simulink model "V3ASM"  (R2020b)
(part 12 of 23)

  Transform63 : sm_lib/Frames and Transforms/Rigid Transform  TranslationMethod=Cartesian  TranslationStandardOffset=0  TranslationLengthUnit=mm  TranslationStandardAxis=+Z  TranslationCartesianOffset=smiData.RigidTransform(303).translation  TranslationROffset=0  TranslationROffsetUnits=m  TranslationZOffset=0  TranslationZOffsetUnits=m  TranslationThetaOffset=0  TranslationThetaOffsetUnits=deg  RotationMethod=ArbitraryAxis  RotationAngleUnits=rad  RotationStandardAxis=+Z  RotationAngle=smiData.RigidTransform(303).angle  RotationArbitraryAxis=smiData.RigidTransform(303).axis  FollAlignAxisA=+X  BaseAlignAxisA=+Y  FollAlignAxisB=+Y  BaseAlignAxisB=+Z  RotationSequenceAxes=FollowerAxes  RotationSequence=XYX  RotationSequenceAngles=[0 0 0]  RotationSequenceAnglesUnits=deg  RotationMatrix=[1 0 0; 0 1 0; 0 0 1]
  Transform64 : sm_lib/Frames and Transforms/Rigid Transform  TranslationMethod=Cartesian  TranslationStandardOffset=0  TranslationLengthUnit=mm  TranslationStandardAxis=+Z  TranslationCartesianOffset=smiData.RigidTransform(304).translation  TranslationROffset=0  TranslationROffsetUnits=m  TranslationZOffset=0  TranslationZOffsetUnits=m  TranslationThetaOffset=0  TranslationThetaOffsetUnits=deg  RotationMethod=ArbitraryAxis  RotationAngleUnits=rad  RotationStandardAxis=+Z  RotationAngle=smiData.RigidTransform(304).angle  RotationArbitraryAxis=smiData.RigidTransform(304).axis  FollAlignAxisA=+X  BaseAlignAxisA=+Y  FollAlignAxisB=+Y  BaseAlignAxisB=+Z  RotationSequenceAxes=FollowerAxes  RotationSequence=XYX  RotationSequenceAngles=[0 0 0]  RotationSequenceAnglesUnits=deg  RotationMatrix=[1 0 0; 0 1 0; 0 0 1]
  Transform65 : sm_lib/Frames and Transforms/Rigid Transform  TranslationMethod=Cartesian  TranslationStandardOffset=0  TranslationLengthUnit=mm  TranslationStandardAxis=+Z  TranslationCartesianOffset=smiData.RigidTransform(305).translation  TranslationROffset=0  TranslationROffsetUnits=m  TranslationZOffset=0  TranslationZOffsetUnits=m  TranslationThetaOffset=0  TranslationThetaOffsetUnits=deg  RotationMethod=ArbitraryAxis  RotationAngleUnits=rad  RotationStandardAxis=+Z  RotationAngle=smiData.RigidTransform(305).angle  RotationArbitraryAxis=smiData.RigidTransform(305).axis  FollAlignAxisA=+X  BaseAlignAxisA=+Y  FollAlignAxisB=+Y  BaseAlignAxisB=+Z  RotationSequenceAxes=FollowerAxes  RotationSequence=XYX  RotationSequenceAngles=[0 0 0]  RotationSequenceAnglesUnits=deg  RotationMatrix=[1 0 0; 0 1 0; 0 0 1]
  Transform66 : sm_lib/Frames and Transforms/Rigid Transform  TranslationMethod=Cartesian  TranslationStandardOffset=0  TranslationLengthUnit=mm  TranslationStandardAxis=+Z  TranslationCartesianOffset=smiData.RigidTransform(306).translation  TranslationROffset=0  TranslationROffsetUnits=m  TranslationZOffset=0  TranslationZOffsetUnits=m  TranslationThetaOffset=0  TranslationThetaOffsetUnits=deg  RotationMethod=ArbitraryAxis  RotationAngleUnits=rad  RotationStandardAxis=+Z  RotationAngle=smiData.RigidTransform(306).angle  RotationArbitraryAxis=smiData.RigidTransform(306).axis  FollAlignAxisA=+X  BaseAlignAxisA=+Y  FollAlignAxisB=+Y  BaseAlignAxisB=+Z  RotationSequenceAxes=FollowerAxes  RotationSequence=XYX  RotationSequenceAngles=[0 0 0]  RotationSequenceAnglesUnits=deg  RotationMatrix=[1 0 0; 0 1 0; 0 0 1]
  Transform67 : sm_lib/Frames and Transforms/Rigid Transform  TranslationMethod=Cartesian  TranslationStandardOffset=0  TranslationLengthUnit=mm  TranslationStandardAxis=+Z  TranslationCartesianOffset=smiData.RigidTransform(307).translation  TranslationROffset=0  TranslationROffsetUnits=m  TranslationZOffset=0  TranslationZOffsetUnits=m  TranslationThetaOffset=0  TranslationThetaOffsetUnits=deg  RotationMethod=ArbitraryAxis  RotationAngleUnits=rad  RotationStandardAxis=+Z  RotationAngle=smiData.RigidTransform(307).angle  RotationArbitraryAxis=smiData.RigidTransform(307).axis  FollAlignAxisA=+X  BaseAlignAxisA=+Y  FollAlignAxisB=+Y  BaseAlignAxisB=+Z  RotationSequenceAxes=FollowerAxes  RotationSequence=XYX  RotationSequenceAngles=[0 0 0]  RotationSequenceAnglesUnits=deg  RotationMatrix=[1 0 0; 0 1 0; 0 0 1]
  Transform68 : sm_lib/Frames and Transforms/Rigid Transform  TranslationMethod=Cartesian  TranslationStandardOffset=0  TranslationLengthUnit=mm  TranslationStandardAxis=+Z  TranslationCartesianOffset=smiData.RigidTransform(308).translation  TranslationROffset=0  TranslationROffsetUnits=m  TranslationZOffset=0  TranslationZOffsetUnits=m  TranslationThetaOffset=0  TranslationThetaOffsetUnits=deg  RotationMethod=ArbitraryAxis  RotationAngleUnits=rad  RotationStandardAxis=+Z  RotationAngle=smiData.RigidTransform(308).angle  RotationArbitraryAxis=smiData.RigidTransform(308).axis  FollAlignAxisA=+X  BaseAlignAxisA=+Y  FollAlignAxisB=+Y  BaseAlignAxisB=+Z  RotationSequenceAxes=FollowerAxes  RotationSequence=XYX  RotationSequenceAngles=[0 0 0]  RotationSequenceAnglesUnits=deg  RotationMatrix=[1 0 0; 0 1 0; 0 0 1]
  Transform69 : sm_lib/Frames and Transforms/Rigid Transform  TranslationMethod=Cartesian  TranslationStandardOffset=0  TranslationLengthUnit=mm  TranslationStandardAxis=+Z  TranslationCartesianOffset=smiData.RigidTransform(309).translation  TranslationROffset=0  TranslationROffsetUnits=m  TranslationZOffset=0  TranslationZOffsetUnits=m  TranslationThetaOffset=0  TranslationThetaOffsetUnits=deg  RotationMethod=ArbitraryAxis  RotationAngleUnits=rad  RotationStandardAxis=+Z  RotationAngle=smiData.RigidTransform(309).angle  RotationArbitraryAxis=smiData.RigidTransform(309).axis  FollAlignAxisA=+X  BaseAlignAxisA=+Y  FollAlignAxisB=+Y  BaseAlignAxisB=+Z  RotationSequenceAxes=FollowerAxes  RotationSequence=XYX  RotationSequenceAngles=[0 0 0]  RotationSequenceAnglesUnits=deg  RotationMatrix=[1 0 0; 0 1 0; 0 0 1]
  Transform7 : sm_lib/Frames and Transforms/Rigid Transform  TranslationMethod=Cartesian  TranslationStandardOffset=0  TranslationLengthUnit=mm  TranslationStandardAxis=+Z  TranslationCartesianOffset=smiData.RigidTransform(247).translation  TranslationROffset=0  TranslationROffsetUnits=m  TranslationZOffset=0  TranslationZOffsetUnits=m  TranslationThetaOffset=0  TranslationThetaOffsetUnits=deg  RotationMethod=ArbitraryAxis  RotationAngleUnits=rad  RotationStandardAxis=+Z  RotationAngle=smiData.RigidTransform(247).angle  RotationArbitraryAxis=smiData.RigidTransform(247).axis  FollAlignAxisA=+X  BaseAlignAxisA=+Y  FollAlignAxisB=+Y  BaseAlignAxisB=+Z  RotationSequenceAxes=FollowerAxes  RotationSequence=XYX  RotationSequenceAngles=[0 0 0]  RotationSequenceAnglesUnits=deg  RotationMatrix=[1 0 0; 0 1 0; 0 0 1]
  Transform70 : sm_lib/Frames and Transforms/Rigid Transform  TranslationMethod=Cartesian  TranslationStandardOffset=0  TranslationLengthUnit=mm  TranslationStandardAxis=+Z  TranslationCartesianOffset=smiData.RigidTransform(310).translation  TranslationROffset=0  TranslationROffsetUnits=m  TranslationZOffset=0  TranslationZOffsetUnits=m  TranslationThetaOffset=0  TranslationThetaOffsetUnits=deg  RotationMethod=ArbitraryAxis  RotationAngleUnits=rad  RotationStandardAxis=+Z  RotationAngle=smiData.RigidTransform(310).angle  RotationArbitraryAxis=smiData.RigidTransform(310).axis  FollAlignAxisA=+X  BaseAlignAxisA=+Y  FollAlignAxisB=+Y  BaseAlignAxisB=+Z  RotationSequenceAxes=FollowerAxes  RotationSequence=XYX  RotationSequenceAngles=[0 0 0]  RotationSequenceAnglesUnits=deg  RotationMatrix=[1 0 0; 0 1 0; 0 0 1]
  Transform71 : sm_lib/Frames and Transforms/Rigid Transform  TranslationMethod=Cartesian  TranslationStandardOffset=0  TranslationLengthUnit=mm  TranslationStandardAxis=+Z  TranslationCartesianOffset=smiData.RigidTransform(311).translation  TranslationROffset=0  TranslationROffsetUnits=m  TranslationZOffset=0  TranslationZOffsetUnits=m  TranslationThetaOffset=0  TranslationThetaOffsetUnits=deg  RotationMethod=ArbitraryAxis  RotationAngleUnits=rad  RotationStandardAxis=+Z  RotationAngle=smiData.RigidTransform(311).angle  RotationArbitraryAxis=smiData.RigidTransform(311).axis  FollAlignAxisA=+X  BaseAlignAxisA=+Y  FollAlignAxisB=+Y  BaseAlignAxisB=+Z  RotationSequenceAxes=FollowerAxes  RotationSequence=XYX  RotationSequenceAngles=[0 0 0]  RotationSequenceAnglesUnits=deg  RotationMatrix=[1 0 0; 0 1 0; 0 0 1]
  Transform72 : sm_lib/Frames and Transforms/Rigid Transform  TranslationMethod=Cartesian  TranslationStandardOffset=0  TranslationLengthUnit=mm  TranslationStandardAxis=+Z  TranslationCartesianOffset=smiData.RigidTransform(312).translation  TranslationROffset=0  TranslationROffsetUnits=m  TranslationZOffset=0  TranslationZOffsetUnits=m  TranslationThetaOffset=0  TranslationThetaOffsetUnits=deg  RotationMethod=ArbitraryAxis  RotationAngleUnits=rad  RotationStandardAxis=+Z  RotationAngle=smiData.RigidTransform(312).angle  RotationArbitraryAxis=smiData.RigidTransform(312).axis  FollAlignAxisA=+X  BaseAlignAxisA=+Y  FollAlignAxisB=+Y  BaseAlignAxisB=+Z  RotationSequenceAxes=FollowerAxes  RotationSequence=XYX  RotationSequenceAngles=[0 0 0]  RotationSequenceAnglesUnits=deg  RotationMatrix=[1 0 0; 0 1 0; 0 0 1]
  Transform73 : sm_lib/Frames and Transforms/Rigid Transform  TranslationMethod=Cartesian  TranslationStandardOffset=0  TranslationLengthUnit=mm  TranslationStandardAxis=+Z  TranslationCartesianOffset=smiData.RigidTransform(313).translation  TranslationROffset=0  TranslationROffsetUnits=m  TranslationZOffset=0  TranslationZOffsetUnits=m  TranslationThetaOffset=0  TranslationThetaOffsetUnits=deg  RotationMethod=ArbitraryAxis  RotationAngleUnits=rad  RotationStandardAxis=+Z  RotationAngle=smiData.RigidTransform(313).angle  RotationArbitraryAxis=smiData.RigidTransform(313).axis  FollAlignAxisA=+X  BaseAlignAxisA=+Y  FollAlignAxisB=+Y  BaseAlignAxisB=+Z  RotationSequenceAxes=FollowerAxes  RotationSequence=XYX  RotationSequenceAngles=[0 0 0]  RotationSequenceAnglesUnits=deg  RotationMatrix=[1 0 0; 0 1 0; 0 0 1]
  Transform74 : sm_lib/Frames and Transforms/Rigid Transform  TranslationMethod=Cartesian  TranslationStandardOffset=0  TranslationLengthUnit=mm  TranslationStandardAxis=+Z  TranslationCartesianOffset=smiData.RigidTransform(314).translation  TranslationROffset=0  TranslationROffsetUnits=m  TranslationZOffset=0  TranslationZOffsetUnits=m  TranslationThetaOffset=0  TranslationThetaOffsetUnits=deg  RotationMethod=ArbitraryAxis  RotationAngleUnits=rad  RotationStandardAxis=+Z  RotationAngle=smiData.RigidTransform(314).angle  RotationArbitraryAxis=smiData.RigidTransform(314).axis  FollAlignAxisA=+X  BaseAlignAxisA=+Y  FollAlignAxisB=+Y  BaseAlignAxisB=+Z  RotationSequenceAxes=FollowerAxes  RotationSequence=XYX  RotationSequenceAngles=[0 0 0]  RotationSequenceAnglesUnits=deg  RotationMatrix=[1 0 0; 0 1 0; 0 0 1]
  Transform75 : sm_lib/Frames and Transforms/Rigid Transform  TranslationMethod=Cartesian  TranslationStandardOffset=0  TranslationLengthUnit=mm  TranslationStandardAxis=+Z  TranslationCartesianOffset=smiData.RigidTransform(315).translation  TranslationROffset=0  TranslationROffsetUnits=m  TranslationZOffset=0  TranslationZOffsetUnits=m  TranslationThetaOffset=0  TranslationThetaOffsetUnits=deg  RotationMethod=ArbitraryAxis  RotationAngleUnits=rad  RotationStandardAxis=+Z  RotationAngle=smiData.RigidTransform(315).angle  RotationArbitraryAxis=smiData.RigidTransform(315).axis  FollAlignAxisA=+X  BaseAlignAxisA=+Y  FollAlignAxisB=+Y  BaseAlignAxisB=+Z  RotationSequenceAxes=FollowerAxes  RotationSequence=XYX  RotationSequenceAngles=[0 0 0]  RotationSequenceAnglesUnits=deg  RotationMatrix=[1 0 0; 0 1 0; 0 0 1]
  Transform76 : sm_lib/Frames and Transforms/Rigid Transform  TranslationMethod=Cartesian  TranslationStandardOffset=0  TranslationLengthUnit=mm  TranslationStandardAxis=+Z  TranslationCartesianOffset=smiData.RigidTransform(316).translation  TranslationROffset=0  TranslationROffsetUnits=m  TranslationZOffset=0  TranslationZOffsetUnits=m  TranslationThetaOffset=0  TranslationThetaOffsetUnits=deg  RotationMethod=ArbitraryAxis  RotationAngleUnits=rad  RotationStandardAxis=+Z  RotationAngle=smiData.RigidTransform(316).angle  RotationArbitraryAxis=smiData.RigidTransform(316).axis  FollAlignAxisA=+X  BaseAlignAxisA=+Y  FollAlignAxisB=+Y  BaseAlignAxisB=+Z  RotationSequenceAxes=FollowerAxes  RotationSequence=XYX  RotationSequenceAngles=[0 0 0]  RotationSequenceAnglesUnits=deg  RotationMatrix=[1 0 0; 0 1 0; 0 0 1]
  Transform77 : sm_lib/Frames and Transforms/Rigid Transform  TranslationMethod=Cartesian  TranslationStandardOffset=0  TranslationLengthUnit=mm  TranslationStandardAxis=+Z  TranslationCartesianOffset=smiData.RigidTransform(317).translation  TranslationROffset=0  TranslationROffsetUnits=m  TranslationZOffset=0  TranslationZOffsetUnits=m  TranslationThetaOffset=0  TranslationThetaOffsetUnits=deg  RotationMethod=ArbitraryAxis  RotationAngleUnits=rad  RotationStandardAxis=+Z  RotationAngle=smiData.RigidTransform(317).angle  RotationArbitraryAxis=smiData.RigidTransform(317).axis  FollAlignAxisA=+X  BaseAlignAxisA=+Y  FollAlignAxisB=+Y  BaseAlignAxisB=+Z  RotationSequenceAxes=FollowerAxes  RotationSequence=XYX  RotationSequenceAngles=[0 0 0]  RotationSequenceAnglesUnits=deg  RotationMatrix=[1 0 0; 0 1 0; 0 0 1]
  Transform78 : sm_lib/Frames and Transforms/Rigid Transform  TranslationMethod=Cartesian  TranslationStandardOffset=0  TranslationLengthUnit=mm  TranslationStandardAxis=+Z  TranslationCartesianOffset=smiData.RigidTransform(318).translation  TranslationROffset=0  TranslationROffsetUnits=m  TranslationZOffset=0  TranslationZOffsetUnits=m  TranslationThetaOffset=0  TranslationThetaOffsetUnits=deg  RotationMethod=ArbitraryAxis  RotationAngleUnits=rad  RotationStandardAxis=+Z  RotationAngle=smiData.RigidTransform(318).angle  RotationArbitraryAxis=smiData.RigidTransform(318).axis  FollAlignAxisA=+X  BaseAlignAxisA=+Y  FollAlignAxisB=+Y  BaseAlignAxisB=+Z  RotationSequenceAxes=FollowerAxes  RotationSequence=XYX  RotationSequenceAngles=[0 0 0]  RotationSequenceAnglesUnits=deg  RotationMatrix=[1 0 0; 0 1 0; 0 0 1]
  Transform79 : sm_lib/Frames and Transforms/Rigid Transform  TranslationMethod=Cartesian  TranslationStandardOffset=0  TranslationLengthUnit=mm  TranslationStandardAxis=+Z  TranslationCartesianOffset=smiData.RigidTransform(319).translation  TranslationROffset=0  TranslationROffsetUnits=m  TranslationZOffset=0  TranslationZOffsetUnits=m  TranslationThetaOffset=0  TranslationThetaOffsetUnits=deg  RotationMethod=ArbitraryAxis  RotationAngleUnits=rad  RotationStandardAxis=+Z  RotationAngle=smiData.RigidTransform(319).angle  RotationArbitraryAxis=smiData.RigidTransform(319).axis  FollAlignAxisA=+X  BaseAlignAxisA=+Y  FollAlignAxisB=+Y  BaseAlignAxisB=+Z  RotationSequenceAxes=FollowerAxes  RotationSequence=XYX  RotationSequenceAngles=[0 0 0]  RotationSequenceAnglesUnits=deg  RotationMatrix=[1 0 0; 0 1 0; 0 0 1]
  Transform8 : sm_lib/Frames and Transforms/Rigid Transform  TranslationMethod=Cartesian  TranslationStandardOffset=0  TranslationLengthUnit=mm  TranslationStandardAxis=+Z  TranslationCartesianOffset=smiData.RigidTransform(248).translation  TranslationROffset=0  TranslationROffsetUnits=m  TranslationZOffset=0  TranslationZOffsetUnits=m  TranslationThetaOffset=0  TranslationThetaOffsetUnits=deg  RotationMethod=ArbitraryAxis  RotationAngleUnits=rad  RotationStandardAxis=+Z  RotationAngle=smiData.RigidTransform(248).angle  RotationArbitraryAxis=smiData.RigidTransform(248).axis  FollAlignAxisA=+X  BaseAlignAxisA=+Y  FollAlignAxisB=+Y  BaseAlignAxisB=+Z  RotationSequenceAxes=FollowerAxes  RotationSequence=XYX  RotationSequenceAngles=[0 0 0]  RotationSequenceAnglesUnits=deg  RotationMatrix=[1 0 0; 0 1 0; 0 0 1]
  Transform80 : sm_lib/Frames and Transforms/Rigid Transform  TranslationMethod=Cartesian  TranslationStandardOffset=0  TranslationLengthUnit=mm  TranslationStandardAxis=+Z  TranslationCartesianOffset=smiData.RigidTransform(320).translation  TranslationROffset=0  TranslationROffsetUnits=m  TranslationZOffset=0  TranslationZOffsetUnits=m  TranslationThetaOffset=0  TranslationThetaOffsetUnits=deg  RotationMethod=ArbitraryAxis  RotationAngleUnits=rad  RotationStandardAxis=+Z  RotationAngle=smiData.RigidTransform(320).angle  RotationArbitraryAxis=smiData.RigidTransform(320).axis  FollAlignAxisA=+X  BaseAlignAxisA=+Y  FollAlignAxisB=+Y  BaseAlignAxisB=+Z  RotationSequenceAxes=FollowerAxes  RotationSequence=XYX  RotationSequenceAngles=[0 0 0]  RotationSequenceAnglesUnits=deg  RotationMatrix=[1 0 0; 0 1 0; 0 0 1]
  Transform81 : sm_lib/Frames and Transforms/Rigid Transform  TranslationMethod=Cartesian  TranslationStandardOffset=0  TranslationLengthUnit=mm  TranslationStandardAxis=+Z  TranslationCartesianOffset=smiData.RigidTransform(321).translation  TranslationROffset=0  TranslationROffsetUnits=m  TranslationZOffset=0  TranslationZOffsetUnits=m  TranslationThetaOffset=0  TranslationThetaOffsetUnits=deg  RotationMethod=ArbitraryAxis  RotationAngleUnits=rad  RotationStandardAxis=+Z  RotationAngle=smiData.RigidTransform(321).angle  RotationArbitraryAxis=smiData.RigidTransform(321).axis  FollAlignAxisA=+X  BaseAlignAxisA=+Y  FollAlignAxisB=+Y  BaseAlignAxisB=+Z  RotationSequenceAxes=FollowerAxes  RotationSequence=XYX  RotationSequenceAngles=[0 0 0]  RotationSequenceAnglesUnits=deg  RotationMatrix=[1 0 0; 0 1 0; 0 0 1]
  Transform82 : sm_lib/Frames and Transforms/Rigid Transform  TranslationMethod=Cartesian  TranslationStandardOffset=0  TranslationLengthUnit=mm  TranslationStandardAxis=+Z  TranslationCartesianOffset=smiData.RigidTransform(322).translation  TranslationROffset=0  TranslationROffsetUnits=m  TranslationZOffset=0  TranslationZOffsetUnits=m  TranslationThetaOffset=0  TranslationThetaOffsetUnits=deg  RotationMethod=ArbitraryAxis  RotationAngleUnits=rad  RotationStandardAxis=+Z  RotationAngle=smiData.RigidTransform(322).angle  RotationArbitraryAxis=smiData.RigidTransform(322).axis  FollAlignAxisA=+X  BaseAlignAxisA=+Y  FollAlignAxisB=+Y  BaseAlignAxisB=+Z  RotationSequenceAxes=FollowerAxes  RotationSequence=XYX  RotationSequenceAngles=[0 0 0]  RotationSequenceAnglesUnits=deg  RotationMatrix=[1 0 0; 0 1 0; 0 0 1]
  Transform83 : sm_lib/Frames and Transforms/Rigid Transform  TranslationMethod=Cartesian  TranslationStandardOffset=0  TranslationLengthUnit=mm  TranslationStandardAxis=+Z  TranslationCartesianOffset=smiData.RigidTransform(323).translation  TranslationROffset=0  TranslationROffsetUnits=m  TranslationZOffset=0  TranslationZOffsetUnits=m  TranslationThetaOffset=0  TranslationThetaOffsetUnits=deg  RotationMethod=ArbitraryAxis  RotationAngleUnits=rad  RotationStandardAxis=+Z  RotationAngle=smiData.RigidTransform(323).angle  RotationArbitraryAxis=smiData.RigidTransform(323).axis  FollAlignAxisA=+X  BaseAlignAxisA=+Y  FollAlignAxisB=+Y  BaseAlignAxisB=+Z  RotationSequenceAxes=FollowerAxes  RotationSequence=XYX  RotationSequenceAngles=[0 0 0]  RotationSequenceAnglesUnits=deg  RotationMatrix=[1 0 0; 0 1 0; 0 0 1]
  Transform84 : sm_lib/Frames and Transforms/Rigid Transform  TranslationMethod=Cartesian  TranslationStandardOffset=0  TranslationLengthUnit=mm  TranslationStandardAxis=+Z  TranslationCartesianOffset=smiData.RigidTransform(324).translation  TranslationROffset=0  TranslationROffsetUnits=m  TranslationZOffset=0  TranslationZOffsetUnits=m  TranslationThetaOffset=0  TranslationThetaOffsetUnits=deg  RotationMethod=ArbitraryAxis  RotationAngleUnits=rad  RotationStandardAxis=+Z  RotationAngle=smiData.RigidTransform(324).angle  RotationArbitraryAxis=smiData.RigidTransform(324).axis  FollAlignAxisA=+X  BaseAlignAxisA=+Y  FollAlignAxisB=+Y  BaseAlignAxisB=+Z  RotationSequenceAxes=FollowerAxes  RotationSequence=XYX  RotationSequenceAngles=[0 0 0]  RotationSequenceAnglesUnits=deg  RotationMatrix=[1 0 0; 0 1 0; 0 0 1]
  Transform85 : sm_lib/Frames and Transforms/Rigid Transform  TranslationMethod=Cartesian  TranslationStandardOffset=0  TranslationLengthUnit=mm  TranslationStandardAxis=+Z  TranslationCartesianOffset=smiData.RigidTransform(325).translation  TranslationROffset=0  TranslationROffsetUnits=m  TranslationZOffset=0  TranslationZOffsetUnits=m  TranslationThetaOffset=0  TranslationThetaOffsetUnits=deg  RotationMethod=ArbitraryAxis  RotationAngleUnits=rad  RotationStandardAxis=+Z  RotationAngle=smiData.RigidTransform(325).angle  RotationArbitraryAxis=smiData.RigidTransform(325).axis  FollAlignAxisA=+X  BaseAlignAxisA=+Y  FollAlignAxisB=+Y  BaseAlignAxisB=+Z  RotationSequenceAxes=FollowerAxes  RotationSequence=XYX  RotationSequenceAngles=[0 0 0]  RotationSequenceAnglesUnits=deg  RotationMatrix=[1 0 0; 0 1 0; 0 0 1]
  Transform86 : sm_lib/Frames and Transforms/Rigid Transform  TranslationMethod=Cartesian  TranslationStandardOffset=0  TranslationLengthUnit=mm  TranslationStandardAxis=+Z  TranslationCartesianOffset=smiData.RigidTransform(326).translation  TranslationROffset=0  TranslationROffsetUnits=m  TranslationZOffset=0  TranslationZOffsetUnits=m  TranslationThetaOffset=0  TranslationThetaOffsetUnits=deg  RotationMethod=ArbitraryAxis  RotationAngleUnits=rad  RotationStandardAxis=+Z  RotationAngle=smiData.RigidTransform(326).angle  RotationArbitraryAxis=smiData.RigidTransform(326).axis  FollAlignAxisA=+X  BaseAlignAxisA=+Y  FollAlignAxisB=+Y  BaseAlignAxisB=+Z  RotationSequenceAxes=FollowerAxes  RotationSequence=XYX  RotationSequenceAngles=[0 0 0]  RotationSequenceAnglesUnits=deg  RotationMatrix=[1 0 0; 0 1 0; 0 0 1]
  Transform87 : sm_lib/Frames and Transforms/Rigid Transform  TranslationMethod=Cartesian  TranslationStandardOffset=0  TranslationLengthUnit=mm  TranslationStandardAxis=+Z  TranslationCartesianOffset=smiData.RigidTransform(327).translation  TranslationROffset=0  TranslationROffsetUnits=m  TranslationZOffset=0  TranslationZOffsetUnits=m  TranslationThetaOffset=0  TranslationThetaOffsetUnits=deg  RotationMethod=ArbitraryAxis  RotationAngleUnits=rad  RotationStandardAxis=+Z  RotationAngle=smiData.RigidTransform(327).angle  RotationArbitraryAxis=smiData.RigidTransform(327).axis  FollAlignAxisA=+X  BaseAlignAxisA=+Y  FollAlignAxisB=+Y  BaseAlignAxisB=+Z  RotationSequenceAxes=FollowerAxes  RotationSequence=XYX  RotationSequenceAngles=[0 0 0]  RotationSequenceAnglesUnits=deg  RotationMatrix=[1 0 0; 0 1 0; 0 0 1]
  Transform88 : sm_lib/Frames and Transforms/Rigid Transform  TranslationMethod=Cartesian  TranslationStandardOffset=0  TranslationLengthUnit=mm  TranslationStandardAxis=+Z  TranslationCartesianOffset=smiData.RigidTransform(328).translation  TranslationROffset=0  TranslationROffsetUnits=m  TranslationZOffset=0  TranslationZOffsetUnits=m  TranslationThetaOffset=0  TranslationThetaOffsetUnits=deg  RotationMethod=ArbitraryAxis  RotationAngleUnits=rad  RotationStandardAxis=+Z  RotationAngle=smiData.RigidTransform(328).angle  RotationArbitraryAxis=smiData.RigidTransform(328).axis  FollAlignAxisA=+X  BaseAlignAxisA=+Y  FollAlignAxisB=+Y  BaseAlignAxisB=+Z  RotationSequenceAxes=FollowerAxes  RotationSequence=XYX  RotationSequenceAngles=[0 0 0]  RotationSequenceAnglesUnits=deg  RotationMatrix=[1 0 0; 0 1 0; 0 0 1]
  Transform89 : sm_lib/Frames and Transforms/Rigid Transform  TranslationMethod=Cartesian  TranslationStandardOffset=0  TranslationLengthUnit=mm  TranslationStandardAxis=+Z  TranslationCartesianOffset=smiData.RigidTransform(329).translation  TranslationROffset=0  TranslationROffsetUnits=m  TranslationZOffset=0  TranslationZOffsetUnits=m  TranslationThetaOffset=0  TranslationThetaOffsetUnits=deg  RotationMethod=ArbitraryAxis  RotationAngleUnits=rad  RotationStandardAxis=+Z  RotationAngle=smiData.RigidTransform(329).angle  RotationArbitraryAxis=smiData.RigidTransform(329).axis  FollAlignAxisA=+X  BaseAlignAxisA=+Y  FollAlignAxisB=+Y  BaseAlignAxisB=+Z  RotationSequenceAxes=FollowerAxes  RotationSequence=XYX  RotationSequenceAngles=[0 0 0]  RotationSequenceAnglesUnits=deg  RotationMatrix=[1 0 0; 0 1 0; 0 0 1]
  Transform9 : sm_lib/Frames and Transforms/Rigid Transform  TranslationMethod=Cartesian  TranslationStandardOffset=0  TranslationLengthUnit=mm  TranslationStandardAxis=+Z  TranslationCartesianOffset=smiData.RigidTransform(249).translation  TranslationROffset=0  TranslationROffsetUnits=m  TranslationZOffset=0  TranslationZOffsetUnits=m  TranslationThetaOffset=0  TranslationThetaOffsetUnits=deg  RotationMethod=ArbitraryAxis  RotationAngleUnits=rad  RotationStandardAxis=+Z  RotationAngle=smiData.RigidTransform(249).angle  RotationArbitraryAxis=smiData.RigidTransform(249).axis  FollAlignAxisA=+X  BaseAlignAxisA=+Y  FollAlignAxisB=+Y  BaseAlignAxisB=+Z  RotationSequenceAxes=FollowerAxes  RotationSequence=XYX  RotationSequenceAngles=[0 0 0]  RotationSequenceAnglesUnits=deg  RotationMatrix=[1 0 0; 0 1 0; 0 0 1]
  Transform90 : sm_lib/Frames and Transforms/Rigid Transform  TranslationMethod=Cartesian  TranslationStandardOffset=0  TranslationLengthUnit=mm  TranslationStandardAxis=+Z  TranslationCartesianOffset=smiData.RigidTransform(330).translation  TranslationROffset=0  TranslationROffsetUnits=m  TranslationZOffset=0  TranslationZOffsetUnits=m  TranslationThetaOffset=0  TranslationThetaOffsetUnits=deg  RotationMethod=ArbitraryAxis  RotationAngleUnits=rad  RotationStandardAxis=+Z  RotationAngle=smiData.RigidTransform(330).angle  RotationArbitraryAxis=smiData.RigidTransform(330).axis  FollAlignAxisA=+X  BaseAlignAxisA=+Y  FollAlignAxisB=+Y  BaseAlignAxisB=+Z  RotationSequenceAxes=FollowerAxes  RotationSequence=XYX  RotationSequenceAngles=[0 0 0]  RotationSequenceAnglesUnits=deg  RotationMatrix=[1 0 0; 0 1 0; 0 0 1]
  Transform91 : sm_lib/Frames and Transforms/Rigid Transform  TranslationMethod=Cartesian  TranslationStandardOffset=0  TranslationLengthUnit=mm  TranslationStandardAxis=+Z  TranslationCartesianOffset=smiData.RigidTransform(331).translation  TranslationROffset=0  TranslationROffsetUnits=m  TranslationZOffset=0  TranslationZOffsetUnits=m  TranslationThetaOffset=0  TranslationThetaOffsetUnits=deg  RotationMethod=ArbitraryAxis  RotationAngleUnits=rad  RotationStandardAxis=+Z  RotationAngle=smiData.RigidTransform(331).angle  RotationArbitraryAxis=smiData.RigidTransform(331).axis  FollAlignAxisA=+X  BaseAlignAxisA=+Y  FollAlignAxisB=+Y  BaseAlignAxisB=+Z  RotationSequenceAxes=FollowerAxes  RotationSequence=XYX  RotationSequenceAngles=[0 0 0]  RotationSequenceAnglesUnits=deg  RotationMatrix=[1 0 0; 0 1 0; 0 0 1]
  Transform92 : sm_lib/Frames and Transforms/Rigid Transform  TranslationMethod=Cartesian  TranslationStandardOffset=0  TranslationLengthUnit=mm  TranslationStandardAxis=+Z  TranslationCartesianOffset=smiData.RigidTransform(332).translation  TranslationROffset=0  TranslationROffsetUnits=m  TranslationZOffset=0  TranslationZOffsetUnits=m  TranslationThetaOffset=0  TranslationThetaOffsetUnits=deg  RotationMethod=ArbitraryAxis  RotationAngleUnits=rad  RotationStandardAxis=+Z  RotationAngle=smiData.RigidTransform(332).angle  RotationArbitraryAxis=smiData.RigidTransform(332).axis  FollAlignAxisA=+X  BaseAlignAxisA=+Y  FollAlignAxisB=+Y  BaseAlignAxisB=+Z  RotationSequenceAxes=FollowerAxes  RotationSequence=XYX  RotationSequenceAngles=[0 0 0]  RotationSequenceAnglesUnits=deg  RotationMatrix=[1 0 0; 0 1 0; 0 0 1]
  Transform93 : sm_lib/Frames and Transforms/Rigid Transform  TranslationMethod=Cartesian  TranslationStandardOffset=0  TranslationLengthUnit=mm  TranslationStandardAxis=+Z  TranslationCartesianOffset=smiData.RigidTransform(333).translation  TranslationROffset=0  TranslationROffsetUnits=m  TranslationZOffset=0  TranslationZOffsetUnits=m  TranslationThetaOffset=0  TranslationThetaOffsetUnits=deg  RotationMethod=ArbitraryAxis  RotationAngleUnits=rad  RotationStandardAxis=+Z  RotationAngle=smiData.RigidTransform(333).angle  RotationArbitraryAxis=smiData.RigidTransform(333).axis  FollAlignAxisA=+X  BaseAlignAxisA=+Y  FollAlignAxisB=+Y  BaseAlignAxisB=+Z  RotationSequenceAxes=FollowerAxes  RotationSequence=XYX  RotationSequenceAngles=[0 0 0]  RotationSequenceAnglesUnits=deg  RotationMatrix=[1 0 0; 0 1 0; 0 0 1]
  Transform94 : sm_lib/Frames and Transforms/Rigid Transform  TranslationMethod=Cartesian  TranslationStandardOffset=0  TranslationLengthUnit=mm  TranslationStandardAxis=+Z  TranslationCartesianOffset=smiData.RigidTransform(334).translation  TranslationROffset=0  TranslationROffsetUnits=m  TranslationZOffset=0  TranslationZOffsetUnits=m  TranslationThetaOffset=0  TranslationThetaOffsetUnits=deg  RotationMethod=ArbitraryAxis  RotationAngleUnits=rad  RotationStandardAxis=+Z  RotationAngle=smiData.RigidTransform(334).angle  RotationArbitraryAxis=smiData.RigidTransform(334).axis  FollAlignAxisA=+X  BaseAlignAxisA=+Y  FollAlignAxisB=+Y  BaseAlignAxisB=+Z  RotationSequenceAxes=FollowerAxes  RotationSequence=XYX  RotationSequenceAngles=[0 0 0]  RotationSequenceAnglesUnits=deg  RotationMatrix=[1 0 0; 0 1 0; 0 0 1]
  Transform95 : sm_lib/Frames and Transforms/Rigid Transform  TranslationMethod=Cartesian  TranslationStandardOffset=0  TranslationLengthUnit=mm  TranslationStandardAxis=+Z  TranslationCartesianOffset=smiData.RigidTransform(335).translation  TranslationROffset=0  TranslationROffsetUnits=m  TranslationZOffset=0  TranslationZOffsetUnits=m  TranslationThetaOffset=0  TranslationThetaOffsetUnits=deg  RotationMethod=ArbitraryAxis  RotationAngleUnits=rad  RotationStandardAxis=+Z  RotationAngle=smiData.RigidTransform(335).angle  RotationArbitraryAxis=smiData.RigidTransform(335).axis  FollAlignAxisA=+X  BaseAlignAxisA=+Y  FollAlignAxisB=+Y  BaseAlignAxisB=+Z  RotationSequenceAxes=FollowerAxes  RotationSequence=XYX  RotationSequenceAngles=[0 0 0]  RotationSequenceAnglesUnits=deg  RotationMatrix=[1 0 0; 0 1 0; 0 0 1]
  Transform96 : sm_lib/Frames and Transforms/Rigid Transform  TranslationMethod=Cartesian  TranslationStandardOffset=0  TranslationLengthUnit=mm  TranslationStandardAxis=+Z  TranslationCartesianOffset=smiData.RigidTransform(336).translation  TranslationROffset=0  TranslationROffsetUnits=m  TranslationZOffset=0  TranslationZOffsetUnits=m  TranslationThetaOffset=0  TranslationThetaOffsetUnits=deg  RotationMethod=ArbitraryAxis  RotationAngleUnits=rad  RotationStandardAxis=+Z  RotationAngle=smiData.RigidTransform(336).angle  RotationArbitraryAxis=smiData.RigidTransform(336).axis  FollAlignAxisA=+X  BaseAlignAxisA=+Y  FollAlignAxisB=+Y  BaseAlignAxisB=+Z  RotationSequenceAxes=FollowerAxes  RotationSequence=XYX  RotationSequenceAngles=[0 0 0]  RotationSequenceAnglesUnits=deg  RotationMatrix=[1 0 0; 0 1 0; 0 0 1]
  Transform97 : sm_lib/Frames and Transforms/Rigid Transform  TranslationMethod=Cartesian  TranslationStandardOffset=0  TranslationLengthUnit=mm  TranslationStandardAxis=+Z  TranslationCartesianOffset=smiData.RigidTransform(337).translation  TranslationROffset=0  TranslationROffsetUnits=m  TranslationZOffset=0  TranslationZOffsetUnits=m  TranslationThetaOffset=0  TranslationThetaOffsetUnits=deg  RotationMethod=ArbitraryAxis  RotationAngleUnits=rad  RotationStandardAxis=+Z  RotationAngle=smiData.RigidTransform(337).angle  RotationArbitraryAxis=smiData.RigidTransform(337).axis  FollAlignAxisA=+X  BaseAlignAxisA=+Y  FollAlignAxisB=+Y  BaseAlignAxisB=+Z  RotationSequenceAxes=FollowerAxes  RotationSequence=XYX  RotationSequenceAngles=[0 0 0]  RotationSequenceAnglesUnits=deg  RotationMatrix=[1 0 0; 0 1 0; 0 0 1]
  Transform98 : sm_lib/Frames and Transforms/Rigid Transform  TranslationMethod=Cartesian  TranslationStandardOffset=0  TranslationLengthUnit=mm  TranslationStandardAxis=+Z  TranslationCartesianOffset=smiData.RigidTransform(338).translation  TranslationROffset=0  TranslationROffsetUnits=m  TranslationZOffset=0  TranslationZOffsetUnits=m  TranslationThetaOffset=0  TranslationThetaOffsetUnits=deg  RotationMethod=ArbitraryAxis  RotationAngleUnits=rad  RotationStandardAxis=+Z  RotationAngle=smiData.RigidTransform(338).angle  RotationArbitraryAxis=smiData.RigidTransform(338).axis  FollAlignAxisA=+X  BaseAlignAxisA=+Y  FollAlignAxisB=+Y  BaseAlignAxisB=+Z  RotationSequenceAxes=FollowerAxes  RotationSequence=XYX  RotationSequenceAngles=[0 0 0]  RotationSequenceAnglesUnits=deg  RotationMatrix=[1 0 0; 0 1 0; 0 0 1]
  Transform99 : sm_lib/Frames and Transforms/Rigid Transform  TranslationMethod=Cartesian  TranslationStandardOffset=0  TranslationLengthUnit=mm  TranslationStandardAxis=+Z  TranslationCartesianOffset=smiData.RigidTransform(339).translation  TranslationROffset=0  TranslationROffsetUnits=m  TranslationZOffset=0  TranslationZOffsetUnits=m  TranslationThetaOffset=0  TranslationThetaOffsetUnits=deg  RotationMethod=ArbitraryAxis  RotationAngleUnits=rad  RotationStandardAxis=+Z  RotationAngle=smiData.RigidTransform(339).angle  RotationArbitraryAxis=smiData.RigidTransform(339).axis  FollAlignAxisA=+X  BaseAlignAxisA=+Y  FollAlignAxisB=+Y  BaseAlignAxisB=+Z  RotationSequenceAxes=FollowerAxes  RotationSequence=XYX  RotationSequenceAngles=[0 0 0]  RotationSequenceAnglesUnits=deg  RotationMatrix=[1 0 0; 0 1 0; 0 0 1]
  VIRTUAL_SHORT_step_10_RIGID : Subsystem
  VIRTUAL_SHORT_step_11_RIGID : Subsystem
  VIRTUAL_SHORT_step_12_RIGID : Subsystem
  VIRTUAL_SHORT_step_13_RIGID : Subsystem
  VIRTUAL_SHORT_step_14_RIGID : Subsystem
  VIRTUAL_SHORT_step_15_RIGID : Subsystem
  VIRTUAL_SHORT_step_16_RIGID : Subsystem
  VIRTUAL_SHORT_step_1_RIGID : Subsystem
  VIRTUAL_SHORT_step_2_RIGID : Subsystem
  VIRTUAL_SHORT_step_3_RIGID : Subsystem
  VIRTUAL_SHORT_step_4_RIGID : Subsystem
  VIRTUAL_SHORT_step_5_RIGID : Subsystem
  VIRTUAL_SHORT_step_6_RIGID : Subsystem
  VIRTUAL_SHORT_step_7_RIGID : Subsystem
  VIRTUAL_SHORT_step_8_RIGID : Subsystem
  VIRTUAL_SHORT_step_9_RIGID : Subsystem
  x032_0256_000_1_step_1_RIGID : Subsystem
  x0402_H040_step_100_RIGID : Subsystem
  x0402_H040_step_101_RIGID : Subsystem
  x0402_H040_step_102_RIGID : Subsystem
  x0402_H040_step_103_RIGID : Subsystem
  x0402_H040_step_104_RIGID : Subsystem
  x0402_H040_step_105_RIGID : Subsystem
  x0402_H040_step_106_RIGID : Subsystem
  x0402_H040_step_107_RIGID : Subsystem
  x0402_H040_step_108_RIGID : Subsystem
  x0402_H040_step_109_RIGID : Subsystem
  x0402_H040_step_10_RIGID : Subsystem
  x0402_H040_step_110_RIGID : Subsystem
  x0402_H040_step_111_RIGID : Subsystem
  x0402_H040_step_112_RIGID : Subsystem
  x0402_H040_step_113_RIGID : Subsystem
  x0402_H040_step_114_RIGID : Subsystem
  x0402_H040_step_115_RIGID : Subsystem
  x0402_H040_step_116_RIGID : Subsystem
  x0402_H040_step_117_RIGID : Subsystem
  x0402_H040_step_118_RIGID : Subsystem
  x0402_H040_step_119_RIGID : Subsystem
  x0402_H040_step_11_RIGID : Subsystem
  x0402_H040_step_120_RIGID : Subsystem
  x0402_H040_step_121_RIGID : Subsystem
  x0402_H040_step_122_RIGID : Subsystem
  x0402_H040_step_123_RIGID : Subsystem
  x0402_H040_step_124_RIGID : Subsystem
  x0402_H040_step_125_RIGID : Subsystem
  x0402_H040_step_126_RIGID : Subsystem
  x0402_H040_step_127_RIGID : Subsystem
  x0402_H040_step_128_RIGID : Subsystem
  x0402_H040_step_129_RIGID : Subsystem
  x0402_H040_step_12_RIGID : Subsystem
  x0402_H040_step_130_RIGID : Subsystem
  x0402_H040_step_131_RIGID : Subsystem
  x0402_H040_step_132_RIGID : Subsystem
  x0402_H040_step_133_RIGID : Subsystem
  x0402_H040_step_134_RIGID : Subsystem
  x0402_H040_step_135_RIGID : Subsystem
  x0402_H040_step_136_RIGID : Subsystem
  x0402_H040_step_137_RIGID : Subsystem
  x0402_H040_step_138_RIGID : Subsystem
  x0402_H040_step_139_RIGID : Subsystem
  x0402_H040_step_13_RIGID : Subsystem
  x0402_H040_step_140_RIGID : Subsystem
  x0402_H040_step_141_RIGID : Subsystem
  x0402_H040_step_142_RIGID : Subsystem
  x0402_H040_step_143_RIGID : Subsystem
  x0402_H040_step_144_RIGID : Subsystem
  x0402_H040_step_145_RIGID : Subsystem
  x0402_H040_step_146_RIGID : Subsystem
  x0402_H040_step_147_RIGID : Subsystem
  x0402_H040_step_148_RIGID : Subsystem
  x0402_H040_step_149_RIGID : Subsystem
  x0402_H040_step_14_RIGID : Subsystem
  x0402_H040_step_15_RIGID : Subsystem
  x0402_H040_step_16_RIGID : Subsystem
  x0402_H040_step_17_RIGID : Subsystem
  x0402_H040_step_18_RIGID : Subsystem
  x0402_H040_step_19_RIGID : Subsystem
  x0402_H040_step_1_RIGID : Subsystem
  x0402_H040_step_20_RIGID : Subsystem
  x0402_H040_step_21_RIGID : Subsystem
  x0402_H040_step_22_RIGID : Subsystem
  x0402_H040_step_23_RIGID : Subsystem
  x0402_H040_step_24_RIGID : Subsystem
  x0402_H040_step_25_RIGID : Subsystem
  x0402_H040_step_26_RIGID : Subsystem
  x0402_H040_step_27_RIGID : Subsystem
  x0402_H040_step_28_RIGID : Subsystem
  x0402_H040_step_29_RIGID : Subsystem
  x0402_H040_step_2_RIGID : Subsystem
  x0402_H040_step_30_RIGID : Subsystem
  x0402_H040_step_31_RIGID : Subsystem
  x0402_H040_step_32_RIGID : Subsystem
  x0402_H040_step_33_RIGID : Subsystem
  x0402_H040_step_34_RIGID : Subsystem
  x0402_H040_step_35_RIGID : Subsystem
  x0402_H040_step_36_RIGID : Subsystem
  x0402_H040_step_37_RIGID : Subsystem
  x0402_H040_step_38_RIGID : Subsystem
  x0402_H040_step_39_RIGID : Subsystem
  x0402_H040_step_3_RIGID : Subsystem
  x0402_H040_step_40_RIGID : Subsystem
  x0402_H040_step_41_RIGID : Subsystem
  x0402_H040_step_42_RIGID : Subsystem
  x0402_H040_step_43_RIGID : Subsystem
  x0402_H040_step_44_RIGID : Subsystem
  x0402_H040_step_45_RIGID : Subsystem
  x0402_H040_step_46_RIGID : Subsystem
  x0402_H040_step_47_RIGID : Subsystem
  x0402_H040_step_48_RIGID : Subsystem
  x0402_H040_step_49_RIGID : Subsystem
  x0402_H040_step_4_RIGID : Subsystem
  x0402_H040_step_50_RIGID : Subsystem
  x0402_H040_step_51_RIGID : Subsystem
  x0402_H040_step_52_RIGID : Subsystem
  x0402_H040_step_53_RIGID : Subsystem
  x0402_H040_step_54_RIGID : Subsystem
  x0402_H040_step_55_RIGID : Subsystem
  x0402_H040_step_56_RIGID : Subsystem
  x0402_H040_step_57_RIGID : Subsystem
  x0402_H040_step_58_RIGID : Subsystem
  x0402_H040_step_59_RIGID : Subsystem
  x0402_H040_step_5_RIGID : Subsystem
  x0402_H040_step_60_RIGID : Subsystem
  x0402_H040_step_61_RIGID : Subsystem
  x0402_H040_step_62_RIGID : Subsystem
  x0402_H040_step_63_RIGID : Subsystem
  x0402_H040_step_64_RIGID : Subsystem
  x0402_H040_step_65_RIGID : Subsystem
  x0402_H040_step_66_RIGID : Subsystem
  x0402_H040_step_67_RIGID : Subsystem
  x0402_H040_step_68_RIGID : Subsystem
  x0402_H040_step_69_RIGID : Subsystem
  x0402_H040_step_6_RIGID : Subsystem
  x0402_H040_step_70_RIGID : Subsystem
  x0402_H040_step_71_RIGID : Subsystem
  x0402_H040_step_72_RIGID : Subsystem
  x0402_H040_step_73_RIGID : Subsystem
  x0402_H040_step_74_RIGID : Subsystem
  x0402_H040_step_75_RIGID : Subsystem
  x0402_H040_step_76_RIGID : Subsystem
  x0402_H040_step_77_RIGID : Subsystem
  x0402_H040_step_78_RIGID : Subsystem
  x0402_H040_step_79_RIGID : Subsystem
  x0402_H040_step_7_RIGID : Subsystem
  x0402_H040_step_80_RIGID : Subsystem
  x0402_H040_step_81_RIGID : Subsystem
  x0402_H040_step_82_RIGID : Subsystem
  x0402_H040_step_83_RIGID : Subsystem
  x0402_H040_step_84_RIGID : Subsystem
  x0402_H040_step_85_RIGID : Subsystem
  x0402_H040_step_86_RIGID : Subsystem
  x0402_H040_step_87_RIGID : Subsystem
  x0402_H040_step_88_RIGID : Subsystem
  x0402_H040_step_89_RIGID : Subsystem
  x0402_H040_step_8_RIGID : Subsystem
  x0402_H040_step_90_RIGID : Subsystem
  x0402_H040_step_91_RIGID : Subsystem
  x0402_H040_step_92_RIGID : Subsystem
  x0402_H040_step_93_RIGID : Subsystem
  x0402_H040_step_94_RIGID : Subsystem
  x0402_H040_step_95_RIGID : Subsystem
  x0402_H040_step_96_RIGID : Subsystem
  x0402_H040_step_97_RIGID : Subsystem
  x0402_H040_step_98_RIGID : Subsystem
  x0402_H040_step_99_RIGID : Subsystem
  x0402_H040_step_9_RIGID : Subsystem
  x0402_H060_step_10_RIGID : Subsystem
  x0402_H060_step_11_RIGID : Subsystem
  x0402_H060_step_12_RIGID : Subsystem
  x0402_H060_step_13_RIGID : Subsystem
  x0402_H060_step_14_RIGID : Subsystem
  x0402_H060_step_15_RIGID : Subsystem
  x0402_H060_step_16_RIGID : Subsystem
  x0402_H060_step_17_RIGID : Subsystem
  x0402_H060_step_18_RIGID : Subsystem
  x0402_H060_step_19_RIGID : Subsystem
  x0402_H060_step_1_RIGID : Subsystem
  x0402_H060_step_20_RIGID : Subsystem
  x0402_H060_step_21_RIGID : Subsystem
  x0402_H060_step_22_RIGID : Subsystem
  x0402_H060_step_23_RIGID : Subsystem
  x0402_H060_step_24_RIGID : Subsystem
  x0402_H060_step_25_RIGID : Subsystem
  x0402_H060_step_26_RIGID : Subsystem
  x0402_H060_step_27_RIGID : Subsystem
  x0402_H060_step_28_RIGID : Subsystem
  x0402_H060_step_29_RIGID : Subsystem
  x0402_H060_step_2_RIGID : Subsystem
  x0402_H060_step_30_RIGID : Subsystem
  x0402_H060_step_31_RIGID : Subsystem
  x0402_H060_step_32_RIGID : Subsystem
  x0402_H060_step_33_RIGID : Subsystem
  x0402_H060_step_34_RIGID : Subsystem
  x0402_H060_step_35_RIGID : Subsystem
  x0402_H060_step_36_RIGID : Subsystem
  x0402_H060_step_37_RIGID : Subsystem
  x0402_H060_step_38_RIGID : Subsystem
  x0402_H060_step_39_RIGID : Subsystem
  x0402_H060_step_3_RIGID : Subsystem
  x0402_H060_step_40_RIGID : Subsystem
  x0402_H060_step_41_RIGID : Subsystem
  x0402_H060_step_42_RIGID : Subsystem
  x0402_H060_step_43_RIGID : Subsystem
  x0402_H060_step_44_RIGID : Subsystem
  x0402_H060_step_45_RIGID : Subsystem
  x0402_H060_step_46_RIGID : Subsystem
  x0402_H060_step_47_RIGID : Subsystem
  x0402_H060_step_48_RIGID : Subsystem
  x0402_H060_step_49_RIGID : Subsystem
  x0402_H060_step_4_RIGID : Subsystem
  x0402_H060_step_50_RIGID : Subsystem
  x0402_H060_step_51_RIGID : Subsystem
  x0402_H060_step_52_RIGID : Subsystem
  x0402_H060_step_53_RIGID : Subsystem
  x0402_H060_step_54_RIGID : Subsystem
  x0402_H060_step_55_RIGID : Subsystem
  x0402_H060_step_56_RIGID : Subsystem
  x0402_H060_step_57_RIGID : Subsystem
  x0402_H060_step_58_RIGID : Subsystem
  x0402_H060_step_59_RIGID : Subsystem
  x0402_H060_step_5_RIGID : Subsystem
  x0402_H060_step_60_RIGID : Subsystem
  x0402_H060_step_61_RIGID : Subsystem
  x0402_H060_step_62_RIGID : Subsystem
  x0402_H060_step_63_RIGID : Subsystem
  x0402_H060_step_64_RIGID : Subsystem
  x0402_H060_step_65_RIGID : Subsystem
  x0402_H060_step_66_RIGID : Subsystem
  x0402_H060_step_67_RIGID : Subsystem
  x0402_H060_step_68_RIGID : Subsystem
  x0402_H060_step_69_RIGID : Subsystem
  x0402_H060_step_6_RIGID : Subsystem
  x0402_H060_step_70_RIGID : Subsystem
  x0402_H060_step_71_RIGID : Subsystem
  x0402_H060_step_72_RIGID : Subsystem
  x0402_H060_step_73_RIGID : Subsystem
  x0402_H060_step_74_RIGID : Subsystem
  x0402_H060_step_75_RIGID : Subsystem
  x0402_H060_step_76_RIGID : Subsystem
  x0402_H060_step_77_RIGID : Subsystem
  x0402_H060_step_78_RIGID : Subsystem
  x0402_H060_step_79_RIGID : Subsystem
  x0402_H060_step_7_RIGID : Subsystem
  x0402_H060_step_80_RIGID : Subsystem
  x0402_H060_step_81_RIGID : Subsystem
  x0402_H060_step_82_RIGID : Subsystem
  x0402_H060_step_83_RIGID : Subsystem
  x0402_H060_step_84_RIGID : Subsystem
  x0402_H060_step_85_RIGID : Subsystem
  x0402_H060_step_86_RIGID : Subsystem
  x0402_H060_step_87_RIGID : Subsystem
  x0402_H060_step_88_RIGID : Subsystem
  x0402_H060_step_89_RIGID : Subsystem
  x0402_H060_step_8_RIGID : Subsystem
  x0402_H060_step_90_RIGID : Subsystem
  x0402_H060_step_91_RIGID : Subsystem
  x0402_H060_step_92_RIGID : Subsystem
  x0402_H060_step_9_RIGID : Subsystem
  x041_0092_000_1_step_1_RIGID : Subsystem
  x0603_H060_step_1_RIGID : Subsystem
  x0603_H060_step_2_RIGID : Subsystem
  x0603_H060_step_3_RIGID : Subsystem
  x0603_H100_step_10_RIGID : Subsystem
  x0603_H100_step_11_RIGID : Subsystem
  x0603_H100_step_12_RIGID : Subsystem
  x0603_H100_step_13_RIGID : Subsystem
  x0603_H100_step_14_RIGID : Subsystem
  x0603_H100_step_15_RIGID : Subsystem
  x0603_H100_step_16_RIGID : Subsystem
  x0603_H100_step_17_RIGID : Subsystem
  x0603_H100_step_1_RIGID : Subsystem
  x0603_H100_step_2_RIGID : Subsystem
  x0603_H100_step_3_RIGID : Subsystem
  x0603_H100_step_4_RIGID : Subsystem
  x0603_H100_step_5_RIGID : Subsystem
  x0603_H100_step_6_RIGID : Subsystem
  x0603_H100_step_7_RIGID : Subsystem
  x0603_H100_step_8_RIGID : Subsystem
  x0603_H100_step_9_RIGID : Subsystem
  x060_0002_000_1_step_1_RIGID : Subsystem
  x064_0373_000_2_step_1_RIGID : Subsystem
  x064_0374_000_2_step_1_RIGID : Subsystem
  x064_0375_000_2_step_1_RIGID : Subsystem
  x064_0377_000_2_step_1_RIGID : Subsystem
  x064_0400_000_1_step_1_RIGID : Subsystem
  x065_0656_000_2_step_1_RIGID : Subsystem
  x065_0656_000_2_step_2_RIGID : Subsystem
  x074_0102_000_4_step_1_RIGID : Subsystem
  x074_0117_000_2_step_1_RIGID : Subsystem
  x074_0216_000_2_step_1_RIGID : Subsystem
  x074_0221_000_3_step_1_RIGID : Subsystem
  x074_0223_000_2_step_1_RIGID : Subsystem
  x0805_H140_step_1_RIGID : Subsystem
  x0805_H150_step_1_RIGID : Subsystem
  x080_1243_000_3_step_1_RIGID : Subsystem
  x080_1368_000_1_step_1_RIGID : Subsystem
  x080_1656_000_3_step_1_RIGID : Subsystem
  x080_1669_000_2_step_1_RIGID : Subsystem
  x085_0328_000_2_step_1_RIGID : Subsystem
  x090_0096_000_1_step_1_RIGID : Subsystem
  x090_0172_000_1_step_1_RIGID : Subsystem
  x090_0172_000_1_step_2_RIGID : Subsystem
  x090_0231_000_1_step_10_RIGID : Subsystem
  x090_0231_000_1_step_11_RIGID : Subsystem
  x090_0231_000_1_step_1_RIGID : Subsystem
  x090_0231_000_1_step_2_RIGID : Subsystem
  x090_0231_000_1_step_3_RIGID : Subsystem
  x090_0231_000_1_step_4_RIGID : Subsystem
  x090_0231_000_1_step_5_RIGID : Subsystem
  x090_0231_000_1_step_6_RIGID : Subsystem
  x090_0231_000_1_step_7_RIGID : Subsystem
  x090_0231_000_1_step_8_RIGID : Subsystem
  x090_0231_000_1_step_9_RIGID : Subsystem
  x090_0233_000_1_step_1_RIGID : Subsystem
  x090_0243_000_1_step_1_RIGID : Subsystem
  x090_0243_000_1_step_2_RIGID : Subsystem
  x090_0243_000_1_step_3_RIGID : Subsystem
  x090_0243_000_1_step_4_RIGID : Subsystem
  x090_0243_000_1_step_5_RIGID : Subsystem
  x090_0309_000_1_step_1_RIGID : Subsystem
  x091_0022_000_1_step_1_RIGID : Subsystem
  x091_0023_000_1_step_1_RIGID : Subsystem
  x092_0073_000_1_step_1_RIGID : Subsystem
  x102_0037_000_1_step_1_RIGID : Subsystem
  x102_0037_000_1_step_2_RIGID : Subsystem
  x102_0037_000_1_step_3_RIGID : Subsystem
  x102_0037_000_1_step_4_RIGID : Subsystem
  x102_0066_000_2_step_1_RIGID : Subsystem
  x102_0066_000_2_step_2_RIGID : Subsystem
  x102_0066_000_2_step_3_RIGID : Subsystem
  x102_0066_000_2_step_4_RIGID : Subsystem
  x102_0066_000_2_step_5_RIGID : Subsystem
  x102_0066_000_2_step_6_RIGID : Subsystem
  x102_0066_000_2_step_7_RIGID : Subsystem
  x102_0066_000_2_step_8_RIGID : Subsystem
  x115_0138_000_1_step_1_RIGID : Subsystem
  x115_0742_000_2_step_1_RIGID : Subsystem
  x115_0742_000_2_step_2_RIGID : Subsystem
  x115_0836_000_1_step_1_RIGID : Subsystem
  x115_0836_000_1_step_2_RIGID : Subsystem
  x115_1232_000_2_step_1_RIGID : Subsystem
  x115_1821_000_1_step_1_RIGID : Subsystem
  x115_1821_000_1_step_2_RIGID : Subsystem
  x115_1821_000_1_step_3_RIGID : Subsystem
  x115_1921_000_3_step_1_RIGID : Subsystem
  x115_1921_000_3_step_2_RIGID : Subsystem
  x115_1921_000_3_step_3_RIGID : Subsystem
  x115_2177_000_2_step_1_RIGID : Subsystem
  x115_2628_000_3_step_1_RIGID : Subsystem
  x1206_H190_step_1_RIGID : Subsystem
  x1206_H190_step_2_RIGID : Subsystem
  x131_0832_000_2_step_1_RIGID : Subsystem
  x142_13449_1000_A02_step_1_RIGID : Subsystem
  x170_0285_000_1_step_1_RIGID : Subsystem
  x174_0159_000_2_step_1_RIGID : Subsystem
  x2016MM_H100_step_1_RIGID : Subsystem
  x300_0402_000_1_step_1_RIGID : Subsystem
  x300_0560_000_1_step_1_RIGID : Subsystem
  x300_0868_000_3_step_10_RIGID : Subsystem
  x300_0868_000_3_step_11_RIGID : Subsystem
  x300_0868_000_3_step_12_RIGID : Subsystem
  x300_0868_000_3_step_13_RIGID : Subsystem
  x300_0868_000_3_step_1_RIGID : Subsystem
  x300_0868_000_3_step_2_RIGID : Subsystem
  x300_0868_000_3_step_3_RIGID : Subsystem
  x300_0868_000_3_step_4_RIGID : Subsystem
  x300_0868_000_3_step_5_RIGID : Subsystem
  x300_0868_000_3_step_6_RIGID : Subsystem
  x300_0868_000_3_step_7_RIGID : Subsystem
  x300_0868_000_3_step_8_RIGID : Subsystem
  x300_0868_000_3_step_9_RIGID : Subsystem
  x300_0869_000_3_step_1_RIGID : Subsystem
  x315_0620_000_1_step_1_RIGID : Subsystem
  x315_1062_000_1_step_1_RIGID : Subsystem
  x315_1109_000_1_step_1_RIGID : Subsystem
  x316_0697_000_1_step_1_RIGID : Subsystem
  F : PMIOPort  Side=Right
  connections:
  Transform/RConn1 -- x315_1109_000_1_step_1_RIGID/LConn1
  Transform1/RConn1 -- x142_13449_1000_A02_step_1_RIGID/LConn1
  Transform10/RConn1 -- x0402_H060_step_1_RIGID/LConn1
  Transform100/RConn1 -- x0402_H060_step_71_RIGID/LConn1
  Transform101/RConn1 -- x0402_H060_step_60_RIGID/LConn1
  Transform102/RConn1 -- x0402_H060_step_59_RIGID/LConn1
  Transform103/RConn1 -- x0402_H060_step_58_RIGID/LConn1
  Transform104/RConn1 -- x0402_H060_step_61_RIGID/LConn1
  Transform105/RConn1 -- x0402_H060_step_66_RIGID/LConn1
  Transform106/RConn1 -- x0402_H060_step_65_RIGID/LConn1
  Transform107/RConn1 -- x0402_H060_step_67_RIGID/LConn1
  Transform108/RConn1 -- x0402_H060_step_68_RIGID/LConn1
  Transform109/RConn1 -- x0402_H060_step_76_RIGID/LConn1
  Transform11/RConn1 -- x0402_H040_step_6_RIGID/LConn1
  Transform110/RConn1 -- x0402_H060_step_74_RIGID/LConn1
  Transform111/RConn1 -- x0402_H060_step_75_RIGID/LConn1
  Transform112/RConn1 -- x0402_H060_step_54_RIGID/LConn1
  Transform113/RConn1 -- x0402_H060_step_78_RIGID/LConn1
  Transform114/RConn1 -- x0402_H060_step_83_RIGID/LConn1
  Transform115/RConn1 -- x0402_H060_step_84_RIGID/LConn1
  Transform116/RConn1 -- x0402_H040_step_35_RIGID/LConn1
  Transform117/RConn1 -- x0402_H060_step_79_RIGID/LConn1
  Transform118/RConn1 -- x0402_H060_step_82_RIGID/LConn1
  Transform119/RConn1 -- x0402_H040_step_36_RIGID/LConn1
  Transform12/RConn1 -- x0402_H040_step_7_RIGID/LConn1
  Transform120/RConn1 -- x0402_H060_step_81_RIGID/LConn1
  Transform121/RConn1 -- x0402_H040_step_37_RIGID/LConn1
  Transform122/RConn1 -- x0402_H040_step_38_RIGID/LConn1
  Transform123/RConn1 -- x0402_H040_step_39_RIGID/LConn1
  Transform124/RConn1 -- x0402_H040_step_40_RIGID/LConn1
  Transform125/RConn1 -- x0402_H060_step_80_RIGID/LConn1
  Transform126/RConn1 -- x0402_H040_step_43_RIGID/LConn1
  Transform127/RConn1 -- x0402_H040_step_61_RIGID/LConn1
  Transform128/RConn1 -- x0402_H040_step_63_RIGID/LConn1
  Transform129/RConn1 -- x0402_H040_step_54_RIGID/LConn1
  Transform13/RConn1 -- x0402_H040_step_8_RIGID/LConn1
  Transform130/RConn1 -- x0402_H040_step_48_RIGID/LConn1
  Transform131/RConn1 -- x0402_H040_step_52_RIGID/LConn1
  Transform132/RConn1 -- x0402_H040_step_44_RIGID/LConn1
  Transform133/RConn1 -- x0402_H040_step_49_RIGID/LConn1
  Transform134/RConn1 -- x0402_H040_step_53_RIGID/LConn1
  Transform135/RConn1 -- x0402_H040_step_59_RIGID/LConn1
  Transform136/RConn1 -- x0402_H040_step_60_RIGID/LConn1
  Transform137/RConn1 -- x0402_H040_step_67_RIGID/LConn1
  Transform138/RConn1 -- x0402_H040_step_47_RIGID/LConn1
  Transform139/RConn1 -- x0402_H040_step_64_RIGID/LConn1
  Transform14/RConn1 -- x0402_H060_step_7_RIGID/LConn1
  Transform140/RConn1 -- x0402_H040_step_78_RIGID/LConn1
  Transform141/RConn1 -- x0402_H040_step_58_RIGID/LConn1
  Transform142/RConn1 -- x0402_H040_step_42_RIGID/LConn1
  Transform143/RConn1 -- x0402_H040_step_45_RIGID/LConn1
  Transform144/RConn1 -- x0402_H040_step_51_RIGID/LConn1
  Transform145/RConn1 -- x0402_H040_step_46_RIGID/LConn1
  Transform146/RConn1 -- x0402_H040_step_55_RIGID/LConn1
  Transform147/RConn1 -- x0402_H040_step_41_RIGID/LConn1
  Transform148/RConn1 -- x0402_H040_step_50_RIGID/LConn1
  Transform149/RConn1 -- x0402_H040_step_56_RIGID/LConn1
  Transform15/RConn1 -- x0402_H060_step_9_RIGID/LConn1
  Transform150/RConn1 -- x0402_H040_step_57_RIGID/LConn1
  Transform151/RConn1 -- x0402_H040_step_62_RIGID/LConn1
  Transform152/RConn1 -- x0402_H040_step_65_RIGID/LConn1
  Transform153/RConn1 -- x0402_H040_step_66_RIGID/LConn1
  Transform154/RConn1 -- x0402_H040_step_68_RIGID/LConn1
  Transform155/RConn1 -- x0402_H040_step_70_RIGID/LConn1
  Transform156/RConn1 -- x0402_H040_step_71_RIGID/LConn1
  Transform157/RConn1 -- x0402_H040_step_72_RIGID/LConn1
  Transform158/RConn1 -- x0402_H040_step_73_RIGID/LConn1
  Transform159/RConn1 -- x0402_H040_step_69_RIGID/LConn1
  Transform16/RConn1 -- x0402_H040_step_9_RIGID/LConn1
  Transform160/RConn1 -- x0402_H040_step_75_RIGID/LConn1
  Transform161/RConn1 -- x0402_H040_step_76_RIGID/LConn1
  Transform162/RConn1 -- x0402_H040_step_74_RIGID/LConn1
  Transform163/RConn1 -- x0402_H040_step_77_RIGID/LConn1
  Transform164/RConn1 -- x0402_H040_step_89_RIGID/LConn1
  Transform165/RConn1 -- x0402_H040_step_92_RIGID/LConn1
  Transform166/RConn1 -- x0402_H040_step_100_RIGID/LConn1
  Transform167/RConn1 -- x0402_H040_step_95_RIGID/LConn1
  Transform168/RConn1 -- x0402_H040_step_80_RIGID/LConn1
  Transform169/RConn1 -- x0402_H040_step_88_RIGID/LConn1
  Transform17/RConn1 -- x0402_H060_step_5_RIGID/LConn1
  Transform170/RConn1 -- x0402_H040_step_101_RIGID/LConn1
  Transform171/RConn1 -- x0402_H040_step_96_RIGID/LConn1
  Transform172/RConn1 -- x0402_H040_step_82_RIGID/LConn1
  Transform173/RConn1 -- x0402_H040_step_97_RIGID/LConn1
  Transform174/RConn1 -- x0402_H040_step_98_RIGID/LConn1
  Transform175/RConn1 -- x0402_H040_step_87_RIGID/LConn1
  Transform176/RConn1 -- x0402_H040_step_102_RIGID/LConn1
  Transform177/RConn1 -- x0402_H040_step_93_RIGID/LConn1
  Transform178/RConn1 -- x0402_H040_step_103_RIGID/LConn1
  Transform179/RConn1 -- x0402_H040_step_104_RIGID/LConn1
  Transform18/RConn1 -- x0402_H060_step_3_RIGID/LConn1
  Transform180/RConn1 -- x0402_H040_step_85_RIGID/LConn1
  Transform181/RConn1 -- x0402_H040_step_79_RIGID/LConn1
  Transform182/RConn1 -- x0402_H040_step_91_RIGID/LConn1
  Transform183/RConn1 -- x0402_H040_step_99_RIGID/LConn1
  Transform184/RConn1 -- x0402_H040_step_81_RIGID/LConn1
  Transform185/RConn1 -- x0402_H040_step_86_RIGID/LConn1
  Transform186/RConn1 -- x0402_H040_step_84_RIGID/LConn1
  Transform187/RConn1 -- x0402_H040_step_83_RIGID/LConn1
  Transform188/RConn1 -- x0402_H040_step_90_RIGID/LConn1
  Transform189/RConn1 -- x0402_H040_step_94_RIGID/LConn1
  Transform19/RConn1 -- x0402_H060_step_2_RIGID/LConn1
  Transform190/RConn1 -- x0402_H040_step_109_RIGID/LConn1
  Transform191/RConn1 -- x0402_H040_step_118_RIGID/LConn1
  Transform192/RConn1 -- x0402_H060_step_85_RIGID/LConn1
  Transform193/RConn1 -- x0402_H040_step_126_RIGID/LConn1
  Transform194/RConn1 -- x0402_H040_step_107_RIGID/LConn1
  Transform195/RConn1 -- x0402_H040_step_108_RIGID/LConn1
  Transform196/RConn1 -- x0402_H040_step_111_RIGID/LConn1
  Transform197/RConn1 -- x0402_H040_step_119_RIGID/LConn1
  Transform198/RConn1 -- x0402_H040_step_121_RIGID/LConn1
  Transform199/RConn1 -- x0402_H040_step_110_RIGID/LConn1
  Transform2/RConn1 -- x0402_H060_step_8_RIGID/LConn1
  Transform20/RConn1 -- x0402_H060_step_11_RIGID/LConn1
  Transform200/RConn1 -- x0402_H040_step_122_RIGID/LConn1
  Transform201/RConn1 -- x0402_H060_step_88_RIGID/LConn1
  Transform202/RConn1 -- x0402_H040_step_125_RIGID/LConn1
  Transform203/RConn1 -- x0402_H040_step_129_RIGID/LConn1
  Transform204/RConn1 -- x0402_H040_step_123_RIGID/LConn1
  Transform205/RConn1 -- x0402_H040_step_106_RIGID/LConn1
  Transform206/RConn1 -- x0402_H040_step_116_RIGID/LConn1
  Transform207/RConn1 -- x0402_H040_step_114_RIGID/LConn1
  Transform208/RConn1 -- x0402_H040_step_117_RIGID/LConn1
  Transform209/RConn1 -- x0402_H040_step_105_RIGID/LConn1
  Transform21/RConn1 -- x0402_H040_step_1_RIGID/LConn1
  Transform210/RConn1 -- x0402_H040_step_120_RIGID/LConn1
  Transform211/RConn1 -- x0402_H040_step_127_RIGID/LConn1
  Transform212/RConn1 -- x0402_H040_step_115_RIGID/LConn1
  Transform213/RConn1 -- x0402_H040_step_113_RIGID/LConn1
  Transform214/RConn1 -- x0402_H040_step_112_RIGID/LConn1
  Transform215/RConn1 -- x0402_H040_step_124_RIGID/LConn1
  Transform216/RConn1 -- x0402_H040_step_128_RIGID/LConn1
  Transform217/RConn1 -- x0402_H060_step_86_RIGID/LConn1
  Transform218/RConn1 -- x0402_H040_step_130_RIGID/LConn1
  Transform219/RConn1 -- x0402_H040_step_131_RIGID/LConn1
  Transform22/RConn1 -- x0402_H060_step_10_RIGID/LConn1
  Transform220/RConn1 -- x0402_H040_step_132_RIGID/LConn1
  Transform221/RConn1 -- x0402_H060_step_87_RIGID/LConn1
  Transform222/RConn1 -- x0402_H040_step_133_RIGID/LConn1
  Transform223/RConn1 -- x0402_H040_step_134_RIGID/LConn1
  Transform224/RConn1 -- x0402_H040_step_135_RIGID/LConn1
  Transform225/RConn1 -- x0402_H040_step_136_RIGID/LConn1
  Transform226/RConn1 -- x0402_H060_step_89_RIGID/LConn1
  Transform227/RConn1 -- x090_0231_000_1_step_3_RIGID/LConn1
  Transform228/RConn1 -- x090_0231_000_1_step_9_RIGID/LConn1
  Transform229/RConn1 -- x090_0231_000_1_step_2_RIGID/LConn1
  Transform23/RConn1 -- x0402_H040_step_2_RIGID/LConn1
  Transform230/RConn1 -- x115_0742_000_2_step_1_RIGID/LConn1
  MEC_STANDOFF_PTH_620C380P_step_1_RIGID/LConn1 -- Transform231/RConn1
  Transform232/RConn1 -- x115_0836_000_1_step_1_RIGID/LConn1
  Transform233/RConn1 -- x115_0836_000_1_step_2_RIGID/LConn1
  Transform234/RConn1 -- x115_1821_000_1_step_2_RIGID/LConn1
  Transform235/RConn1 -- x080_1656_000_3_step_1_RIGID/LConn1
  Transform236/RConn1 -- x090_0231_000_1_step_1_RIGID/LConn1
  Transform237/RConn1 -- x090_0231_000_1_step_5_RIGID/LConn1
  Transform238/RConn1 -- x090_0231_000_1_step_7_RIGID/LConn1
  Transform239/RConn1 -- x090_0231_000_1_step_10_RIGID/LConn1
  Transform24/RConn1 -- x0402_H040_step_3_RIGID/LConn1
  Transform240/RConn1 -- x090_0231_000_1_step_4_RIGID/LConn1
  Transform241/RConn1 -- x090_0231_000_1_step_6_RIGID/LConn1
  Transform242/RConn1 -- x315_0620_000_1_step_1_RIGID/LConn1
  Transform243/RConn1 -- x074_0102_000_4_step_1_RIGID/LConn1
  Transform244/RConn1 -- x090_0231_000_1_step_8_RIGID/LConn1
  Transform245/RConn1 -- x315_1062_000_1_step_1_RIGID/LConn1
  Transform246/RConn1 -- x090_0231_000_1_step_11_RIGID/LConn1
  Transform247/RConn1 -- x115_1821_000_1_step_1_RIGID/LConn1
  Transform248/RConn1 -- x091_0023_000_1_step_1_RIGID/LConn1
  Transform249/RConn1 -- x074_0223_000_2_step_1_RIGID/LConn1
  Transform25/RConn1 -- x0402_H040_step_17_RIGID/LConn1
  Transform250/RConn1 -- x064_0400_000_1_step_1_RIGID/LConn1
  Transform251/RConn1 -- x131_0832_000_2_step_1_RIGID/LConn1
  Transform252/RConn1 -- x115_0138_000_1_step_1_RIGID/LConn1
  Transform253/RConn1 -- x170_0285_000_1_step_1_RIGID/LConn1
  Transform254/RConn1 -- x115_1821_000_1_step_3_RIGID/LConn1
  Transform255/RConn1 -- x091_0022_000_1_step_1_RIGID/LConn1
  Transform256/RConn1 -- x080_1368_000_1_step_1_RIGID/LConn1
  Transform257/RConn1 -- x300_0868_000_3_step_5_RIGID/LConn1
  Transform258/RConn1 -- x115_0742_000_2_step_2_RIGID/LConn1
  Transform259/RConn1 -- x115_2177_000_2_step_1_RIGID/LConn1
  Transform26/RConn1 -- x0402_H040_step_22_RIGID/LConn1
  Transform260/RConn1 -- x300_0868_000_3_step_7_RIGID/LConn1
  Transform261/RConn1 -- x300_0868_000_3_step_2_RIGID/LConn1
  Transform262/RConn1 -- x300_0868_000_3_step_11_RIGID/LConn1
  IND_SMD_0402_H060_step_1_RIGID/LConn1 -- Transform263/RConn1
  Transform264/RConn1 -- x090_0172_000_1_step_2_RIGID/LConn1
  Transform265/RConn1 -- x1206_H190_step_2_RIGID/LConn1
  Transform266/RConn1 -- x300_0560_000_1_step_1_RIGID/LConn1
  Transform267/RConn1 -- x300_0868_000_3_step_1_RIGID/LConn1
  Transform268/RConn1 -- x090_0243_000_1_step_5_RIGID/LConn1
  Transform269/RConn1 -- x090_0243_000_1_step_1_RIGID/LConn1
  Transform27/RConn1 -- x0402_H040_step_19_RIGID/LConn1
  Transform270/RConn1 -- x090_0233_000_1_step_1_RIGID/LConn1
  Transform271/RConn1 -- x115_2628_000_3_step_1_RIGID/LConn1
  Transform272/RConn1 -- x092_0073_000_1_step_1_RIGID/LConn1
  Transform273/RConn1 -- x090_0243_000_1_step_2_RIGID/LConn1
  Transform274/RConn1 -- x090_0243_000_1_step_3_RIGID/LConn1
  Transform275/RConn1 -- x064_0374_000_2_step_1_RIGID/LConn1
  Transform276/RConn1 -- x090_0243_000_1_step_4_RIGID/LConn1
  Transform277/RConn1 -- x1206_H190_step_1_RIGID/LConn1
  Transform278/RConn1 -- x300_0868_000_3_step_3_RIGID/LConn1
  Transform279/RConn1 -- x300_0868_000_3_step_4_RIGID/LConn1
  Transform28/RConn1 -- x0402_H060_step_20_RIGID/LConn1
  Transform280/RConn1 -- x090_0172_000_1_step_1_RIGID/LConn1
  Transform281/RConn1 -- x300_0868_000_3_step_6_RIGID/LConn1
  Transform282/RConn1 -- x300_0868_000_3_step_8_RIGID/LConn1
  Transform283/RConn1 -- x300_0868_000_3_step_9_RIGID/LConn1
  Transform284/RConn1 -- x300_0868_000_3_step_10_RIGID/LConn1
  Transform285/RConn1 -- x300_0868_000_3_step_12_RIGID/LConn1
  Transform286/RConn1 -- x300_0868_000_3_step_13_RIGID/LConn1
  Transform287/RConn1 -- x300_0869_000_3_step_1_RIGID/LConn1
  Transform288/RConn1 -- x300_0402_000_1_step_1_RIGID/LConn1
  Transform289/RConn1 -- x174_0159_000_2_step_1_RIGID/LConn1
  Transform29/RConn1 -- x0402_H040_step_20_RIGID/LConn1
  Transform290/RConn1 -- x064_0373_000_2_step_1_RIGID/LConn1
  Transform291/RConn1 -- x0402_H060_step_91_RIGID/LConn1
  Transform292/RConn1 -- VIRTUAL_SHORT_step_1_RIGID/LConn1
  Transform293/RConn1 -- VIRTUAL_SHORT_step_2_RIGID/LConn1
  Transform294/RConn1 -- x0402_H040_step_148_RIGID/LConn1
  Transform295/RConn1 -- VIRTUAL_SHORT_step_5_RIGID/LConn1
  Transform296/RConn1 -- x0402_H040_step_147_RIGID/LConn1
  Transform297/RConn1 -- VIRTUAL_SHORT_step_12_RIGID/LConn1
  Transform298/RConn1 -- VIRTUAL_SHORT_step_15_RIGID/LConn1
  Transform299/RConn1 -- VIRTUAL_SHORT_step_14_RIGID/LConn1
  Transform3/RConn1 -- x0402_H040_step_10_RIGID/LConn1
  Transform30/RConn1 -- x0402_H040_step_25_RIGID/LConn1
  Transform300/RConn1 -- x0402_H060_step_92_RIGID/LConn1
  Transform301/RConn1 -- VIRTUAL_SHORT_step_4_RIGID/LConn1
  Transform302/RConn1 -- x0402_H060_step_90_RIGID/LConn1
  Transform303/RConn1 -- x0402_H040_step_149_RIGID/LConn1
  Transform304/RConn1 -- VIRTUAL_SHORT_step_7_RIGID/LConn1
  Transform305/RConn1 -- x0402_H040_step_137_RIGID/LConn1
  Transform306/RConn1 -- VIRTUAL_SHORT_step_3_RIGID/LConn1
  Transform307/RConn1 -- x0402_H040_step_144_RIGID/LConn1
  Transform308/RConn1 -- x0402_H040_step_141_RIGID/LConn1
  Transform309/RConn1 -- x0402_H040_step_140_RIGID/LConn1
  Transform31/RConn1 -- x0402_H040_step_16_RIGID/LConn1
  Transform310/RConn1 -- x0402_H040_step_142_RIGID/LConn1
  Transform311/RConn1 -- x0402_H040_step_146_RIGID/LConn1
  Transform312/RConn1 -- x0402_H040_step_138_RIGID/LConn1
  Transform313/RConn1 -- x0402_H040_step_139_RIGID/LConn1
  Transform314/RConn1 -- x0402_H040_step_143_RIGID/LConn1
  Transform315/RConn1 -- x0402_H040_step_145_RIGID/LConn1
  Transform316/RConn1 -- VIRTUAL_SHORT_step_6_RIGID/LConn1
  Transform317/RConn1 -- VIRTUAL_SHORT_step_8_RIGID/LConn1
  Transform318/RConn1 -- VIRTUAL_SHORT_step_9_RIGID/LConn1
  Transform319/RConn1 -- VIRTUAL_SHORT_step_10_RIGID/LConn1
  Transform32/RConn1 -- x0402_H060_step_23_RIGID/LConn1
  Transform320/RConn1 -- VIRTUAL_SHORT_step_11_RIGID/LConn1
  Transform321/RConn1 -- VIRTUAL_SHORT_step_13_RIGID/LConn1
  Transform322/RConn1 -- VIRTUAL_SHORT_step_16_RIGID/LConn1
  Transform323/RConn1 -- x064_0377_000_2_step_1_RIGID/LConn1
  Transform324/RConn1 -- x074_0117_000_2_step_1_RIGID/LConn1
  Transform325/RConn1 -- x090_0096_000_1_step_1_RIGID/LConn1
  Transform326/RConn1 -- x090_0309_000_1_step_1_RIGID/LConn1
  Transform327/RConn1 -- x115_1232_000_2_step_1_RIGID/LConn1
  Transform328/RConn1 -- x316_0697_000_1_step_1_RIGID/LConn1
  Transform329/RConn1 -- x060_0002_000_1_step_1_RIGID/LConn1
  Transform33/RConn1 -- x0402_H040_step_13_RIGID/LConn1
  Transform330/RConn1 -- x102_0037_000_1_step_2_RIGID/LConn1
  Transform331/RConn1 -- x102_0066_000_2_step_7_RIGID/LConn1
  Transform332/RConn1 -- x0805_H140_step_1_RIGID/LConn1
  Transform333/RConn1 -- x102_0066_000_2_step_8_RIGID/LConn1
  Transform334/RConn1 -- x102_0066_000_2_step_6_RIGID/LConn1
  Transform335/RConn1 -- x102_0066_000_2_step_2_RIGID/LConn1
  Transform336/RConn1 -- x080_1243_000_3_step_1_RIGID/LConn1
  Transform337/RConn1 -- x115_1921_000_3_step_3_RIGID/LConn1
  Transform338/RConn1 -- x102_0066_000_2_step_1_RIGID/LConn1
  Transform339/RConn1 -- x074_0216_000_2_step_1_RIGID/LConn1
  Transform34/RConn1 -- x0402_H040_step_15_RIGID/LConn1
  Transform340/RConn1 -- x074_0221_000_3_step_1_RIGID/LConn1
  Transform341/RConn1 -- x115_1921_000_3_step_2_RIGID/LConn1
  Transform342/RConn1 -- x2016MM_H100_step_1_RIGID/LConn1
  Transform343/RConn1 -- x065_0656_000_2_step_2_RIGID/LConn1
  Transform344/RConn1 -- x115_1921_000_3_step_1_RIGID/LConn1
  Transform345/RConn1 -- x032_0256_000_1_step_1_RIGID/LConn1
  Transform346/RConn1 -- x041_0092_000_1_step_1_RIGID/LConn1
  Transform347/RConn1 -- x064_0375_000_2_step_1_RIGID/LConn1
  Transform348/RConn1 -- x065_0656_000_2_step_1_RIGID/LConn1
  Transform349/RConn1 -- x085_0328_000_2_step_1_RIGID/LConn1
  Transform35/RConn1 -- x0402_H060_step_24_RIGID/LConn1
  Transform350/RConn1 -- x102_0066_000_2_step_4_RIGID/LConn1
  Transform351/RConn1 -- x102_0066_000_2_step_3_RIGID/LConn1
  Transform352/RConn1 -- x102_0066_000_2_step_5_RIGID/LConn1
  Transform353/RConn1 -- x102_0037_000_1_step_1_RIGID/LConn1
  Transform354/RConn1 -- x102_0037_000_1_step_3_RIGID/LConn1
  Transform355/RConn1 -- x102_0037_000_1_step_4_RIGID/LConn1
  Transform356/RConn1 -- x0603_H100_step_6_RIGID/LConn1
  Transform357/RConn1 -- x0603_H100_step_7_RIGID/LConn1
  Transform358/RConn1 -- x0603_H060_step_1_RIGID/LConn1
  Transform359/RConn1 -- x0603_H100_step_13_RIGID/LConn1
  Transform36/RConn1 -- x0402_H040_step_12_RIGID/LConn1
  Transform360/RConn1 -- x0603_H060_step_3_RIGID/LConn1
  Transform361/RConn1 -- x0603_H100_step_3_RIGID/LConn1
  Transform362/RConn1 -- x0603_H100_step_8_RIGID/LConn1
  Transform363/RConn1 -- x0603_H100_step_1_RIGID/LConn1
  Transform364/RConn1 -- x0603_H100_step_16_RIGID/LConn1
  Transform365/RConn1 -- x0603_H100_step_15_RIGID/LConn1
  Transform366/RConn1 -- x0603_H100_step_2_RIGID/LConn1
  Transform367/RConn1 -- x080_1669_000_2_step_1_RIGID/LConn1
  Transform368/RConn1 -- x0805_H150_step_1_RIGID/LConn1
  Transform369/RConn1 -- x0603_H100_step_4_RIGID/LConn1
  Transform37/RConn1 -- x0402_H060_step_17_RIGID/LConn1
  Transform370/RConn1 -- x0603_H100_step_11_RIGID/LConn1
  Transform371/RConn1 -- x0603_H100_step_5_RIGID/LConn1
  Transform372/RConn1 -- x0603_H060_step_2_RIGID/LConn1
  Transform373/RConn1 -- x0603_H100_step_9_RIGID/LConn1
  Transform374/RConn1 -- x0603_H100_step_12_RIGID/LConn1
  Transform375/RConn1 -- x0603_H100_step_17_RIGID/LConn1
  Transform376/RConn1 -- x0603_H100_step_10_RIGID/LConn1
  Transform377/RConn1 -- x0603_H100_step_14_RIGID/LConn1
  Transform/LConn1 -- ReferenceFrame/RConn1 -- Transform1/LConn1 -- Transform10/LConn1 -- Transform100/LConn1 -- Transform101/LConn1 -- Transform102/LConn1 -- Transform103/LConn1 -- Transform104/LConn1 -- Transform105/LConn1 -- Transform106/LConn1 -- Transform107/LConn1 -- Transform108/LConn1 -- Transform109/LConn1 -- Transform11/LConn1 -- Transform110/LConn1 -- Transform111/LConn1 -- Transform112/LConn1 -- Transform113/LConn1 -- Transform114/LConn1 -- Transform115/LConn1 -- Transform116/LConn1 -- Transform117/LConn1 -- Transform118/LConn1 -- Transform119/LConn1 -- Transform12/LConn1 -- Transform120/LConn1 -- Transform121/LConn1 -- Transform122/LConn1 -- Transform123/LConn1 -- Transform124/LConn1 -- Transform125/LConn1 -- Transform126/LConn1 -- Transform127/LConn1 -- Transform128/LConn1 -- Transform129/LConn1 -- Transform13/LConn1 -- Transform130/LConn1 -- Transform131/LConn1 -- Transform132/LConn1 -- Transform133/LConn1 -- Transform134/LConn1 -- Transform135/LConn1 -- Transform136/LConn1 -- Transform137/LConn1 -- Transform138/LConn1 -- Transform139/LConn1 -- Transform14/LConn1 -- Transform140/LConn1 -- Transform141/LConn1 -- Transform142/LConn1 -- Transform143/LConn1 -- Transform144/LConn1 -- Transform145/LConn1 -- Transform146/LConn1 -- Transform147/LConn1 -- Transform148/LConn1 -- Transform149/LConn1 -- Transform15/LConn1 -- Transform150/LConn1 -- Transform151/LConn1 -- Transform152/LConn1 -- Transform153/LConn1 -- Transform154/LConn1 -- Transform155/LConn1 -- Transform156/LConn1 -- Transform157/LConn1 -- Transform158/LConn1 -- Transform159/LConn1 -- Transform16/LConn1 -- Transform160/LConn1 -- Transform161/LConn1 -- Transform162/LConn1 -- Transform163/LConn1 -- Transform164/LConn1 -- Transform165/LConn1 -- Transform166/LConn1 -- Transform167/LConn1 -- Transform168/LConn1 -- Transform169/LConn1 -- Transform17/LConn1 -- Transform170/LConn1 -- Transform171/LConn1 -- Transform172/LConn1 -- Transform173/LConn1 -- Transform174/LConn1 -- Transform175/LConn1 -- Transform176/LConn1 -- Transform177/LConn1 -- Transform178/LConn1 -- Transform179/LConn1 -- Transform18/LConn1 -- Transform180/LConn1 -- Transform181/LConn1 -- Transform182/LConn1 -- Transform183/LConn1 -- Transform184/LConn1 -- Transform185/LConn1 -- Transform186/LConn1 -- Transform187/LConn1 -- Transform188/LConn1 -- Transform189/LConn1 -- Transform19/LConn1 -- Transform190/LConn1 -- Transform191/LConn1 -- Transform192/LConn1 -- Transform193/LConn1 -- Transform194/LConn1 -- Transform195/LConn1 -- Transform196/LConn1 -- Transform197/LConn1 -- Transform198/LConn1 -- Transform199/LConn1 -- Transform2/LConn1 -- Transform20/LConn1 -- Transform200/LConn1 -- Transform201/LConn1 -- Transform202/LConn1 -- Transform203/LConn1 -- Transform204/LConn1 -- Transform205/LConn1 -- Transform206/LConn1 -- Transform207/LConn1 -- Transform208/LConn1 -- Transform209/LConn1 -- Transform21/LConn1 -- Transform210/LConn1 -- Transform211/LConn1 -- Transform212/LConn1 -- Transform213/LConn1 -- Transform214/LConn1 -- Transform215/LConn1 -- Transform216/LConn1 -- Transform217/LConn1 -- Transform218/LConn1 -- Transform219/LConn1 -- Transform22/LConn1 -- Transform220/LConn1 -- Transform221/LConn1 -- Transform222/LConn1 -- Transform223/LConn1 -- Transform224/LConn1 -- Transform225/LConn1 -- Transform226/LConn1 -- Transform227/LConn1 -- Transform228/LConn1 -- Transform229/LConn1 -- Transform23/LConn1 -- Transform230/LConn1 -- Transform231/LConn1 -- Transform232/LConn1 -- Transform233/LConn1 -- Transform234/LConn1 -- Transform235/LConn1 -- Transform236/LConn1 -- Transform237/LConn1 -- Transform238/LConn1 -- Transform239/LConn1 -- Transform24/LConn1 -- Transform240/LConn1 -- Transform241/LConn1 -- Transform242/LConn1 -- Transform243/LConn1 -- Transform244/LConn1 -- Transform245/LConn1 -- Transform246/LConn1 -- Transform247/LConn1 -- Transform248/LConn1 -- Transform249/LConn1 -- Transform25/LConn1 -- Transform250/LConn1 -- Transform251/LConn1 -- Transform252/LConn1 -- Transform253/LConn1 -- Transform254/LConn1 -- Transform255/LConn1 -- Transform256/LConn1 -- Transform257/LConn1 -- Transform258/LConn1 -- Transform259/LConn1 -- Transform26/LConn1 -- Transform260/LConn1 -- Transform261/LConn1 -- Transform262/LConn1 -- Transform263/LConn1 -- Transform264/LConn1 -- Transform265/LConn1 -- Transform266/LConn1 -- Transform267/LConn1 -- Transform268/LConn1 -- Transform269/LConn1 -- Transform27/LConn1 -- Transform270/LConn1 -- Transform271/LConn1 -- Transform272/LConn1 -- Transform273/LConn1 -- Transform274/LConn1 -- Transform275/LConn1 -- Transform276/LConn1 -- Transform277/LConn1 -- Transform278/LConn1 -- Transform279/LConn1 -- Transform28/LConn1 -- Transform280/LConn1 -- Transform281/LConn1 -- Transform282/LConn1 -- Transform283/LConn1 -- Transform284/LConn1 -- Transform285/LConn1 -- Transform286/LConn1 -- Transform287/LConn1 -- Transform288/LConn1 -- Transform289/LConn1 -- Transform29/LConn1 -- Transform290/LConn1 -- Transform291/LConn1 -- Transform292/LConn1 -- Transform293/LConn1 -- Transform294/LConn1 -- Transform295/LConn1 -- Transform296/LConn1 -- Transform297/LConn1 -- Transform298/LConn1 -- Transform299/LConn1 -- Transform3/LConn1 -- Transform30/LConn1 -- Transform300/LConn1 -- Transform301/LConn1 -- Transform302/LConn1 -- Transform303/LConn1 -- Transform304/LConn1 -- Transform305/LConn1 -- Transform306/LConn1 -- Transform307/LConn1 -- Transform308/LConn1 -- Transform309/LConn1 -- Transform31/LConn1 -- Transform310/LConn1 -- Transform311/LConn1 -- Transform312/LConn1 -- Transform313/LConn1 -- Transform314/LConn1 -- Transform315/LConn1 -- Transform316/LConn1 -- Transform317/LConn1 -- Transform318/LConn1 -- Transform319/LConn1 -- Transform32/LConn1 -- Transform320/LConn1 -- Transform321/LConn1 -- Transform322/LConn1 -- Transform323/LConn1 -- Transform324/LConn1 -- Transform325/LConn1 -- Transform326/LConn1 -- Transform327/LConn1 -- Transform328/LConn1 -- Transform329/LConn1 -- Transform33/LConn1 -- Transform330/LConn1 -- Transform331/LConn1 -- Transform332/LConn1 -- Transform333/LConn1 -- Transform334/LConn1 -- Transform335/LConn1 -- Transform336/LConn1 -- Transform337/LConn1 -- Transform338/LConn1 -- Transform339/LConn1 -- Transform34/LConn1 -- Transform340/LConn1 -- Transform341/LConn1 -- Transform342/LConn1 -- Transform343/LConn1 -- Transform344/LConn1 -- Transform345/LConn1 -- Transform346/LConn1 -- Transform347/LConn1 -- Transform348/LConn1 -- Transform349/LConn1 -- Transform35/LConn1 -- Transform350/LConn1 -- Transform351/LConn1 -- Transform352/LConn1 -- Transform353/LConn1 -- Transform354/LConn1 -- Transform355/LConn1 -- Transform356/LConn1 -- Transform357/LConn1 -- Transform358/LConn1 -- Transform359/LConn1 -- Transform36/LConn1 -- Transform360/LConn1 -- Transform361/LConn1 -- Transform362/LConn1 -- Transform363/LConn1 -- Transform364/LConn1 -- Transform365/LConn1 -- Transform366/LConn1 -- Transform367/LConn1 -- Transform368/LConn1 -- Transform369/LConn1 -- Transform37/LConn1 -- Transform370/LConn1 -- Transform371/LConn1 -- Transform372/LConn1 -- Transform373/LConn1 -- Transform374/LConn1 -- Transform375/LConn1 -- Transform376/LConn1 -- Transform377/LConn1 -- Transform378/RConn1 -- Transform38/LConn1 -- Transform39/LConn1 -- Transform4/LConn1 -- Transform40/LConn1 -- Transform41/LConn1 -- Transform42/LConn1 -- Transform43/LConn1 -- Transform44/LConn1 -- Transform45/LConn1 -- Transform46/LConn1 -- Transform47/LConn1 -- Transform48/LConn1 -- Transform49/LConn1 -- Transform5/LConn1 -- Transform50/LConn1 -- Transform51/LConn1 -- Transform52/LConn1 -- Transform53/LConn1 -- Transform54/LConn1 -- Transform55/LConn1 -- Transform56/LConn1 -- Transform57/LConn1 -- Transform58/LConn1 -- Transform59/LConn1 -- Transform6/LConn1 -- Transform60/LConn1 -- Transform61/LConn1 -- Transform62/LConn1 -- Transform63/LConn1 -- Transform64/LConn1 -- Transform65/LConn1 -- Transform66/LConn1 -- Transform67/LConn1 -- Transform68/LConn1 -- Transform69/LConn1 -- Transform7/LConn1 -- Transform70/LConn1 -- Transform71/LConn1 -- Transform72/LConn1 -- Transform73/LConn1 -- Transform74/LConn1 -- Transform75/LConn1 -- Transform76/LConn1 -- Transform77/LConn1 -- Transform78/LConn1 -- Transform79/LConn1 -- Transform8/LConn1 -- Transform80/LConn1 -- Transform81/LConn1 -- Transform82/LConn1 -- Transform83/LConn1 -- Transform84/LConn1 -- Transform85/LConn1 -- Transform86/LConn1 -- Transform87/LConn1 -- Transform88/LConn1 -- Transform89/LConn1 -- Transform9/LConn1 -- Transform90/LConn1 -- Transform91/LConn1 -- Transform92/LConn1 -- Transform93/LConn1 -- Transform94/LConn1 -- Transform95/LConn1 -- Transform96/LConn1 -- Transform97/LConn1 -- Transform98/LConn1 -- Transform99/LConn1
  Transform378/LConn1 -- F/RConn1
  Transform38/RConn1 -- x0402_H040_step_18_RIGID/LConn1
  Transform39/RConn1 -- x0402_H060_step_15_RIGID/LConn1
  Transform4/RConn1 -- x0402_H040_step_11_RIGID/LConn1
  Transform40/RConn1 -- x0402_H060_step_18_RIGID/LConn1
  Transform41/RConn1 -- x0402_H060_step_19_RIGID/LConn1
  Transform42/RConn1 -- x0402_H060_step_13_RIGID/LConn1
  Transform43/RConn1 -- x0402_H060_step_22_RIGID/LConn1
  Transform44/RConn1 -- x0402_H060_step_25_RIGID/LConn1
  Transform45/RConn1 -- x0402_H040_step_14_RIGID/LConn1
  Transform46/RConn1 -- x0402_H060_step_16_RIGID/LConn1
  Transform47/RConn1 -- x0402_H060_step_21_RIGID/LConn1
  Transform48/RConn1 -- x0402_H060_step_14_RIGID/LConn1
  Transform49/RConn1 -- x0402_H040_step_21_RIGID/LConn1
  Transform5/RConn1 -- x0402_H060_step_12_RIGID/LConn1
  Transform50/RConn1 -- x0402_H060_step_27_RIGID/LConn1
  Transform51/RConn1 -- x0402_H040_step_23_RIGID/LConn1
  Transform52/RConn1 -- x0402_H040_step_24_RIGID/LConn1
  Transform53/RConn1 -- x0402_H060_step_26_RIGID/LConn1
  Transform54/RConn1 -- x0402_H060_step_29_RIGID/LConn1
  Transform55/RConn1 -- x0402_H040_step_27_RIGID/LConn1
  Transform56/RConn1 -- x0402_H060_step_39_RIGID/LConn1
  Transform57/RConn1 -- x0402_H060_step_42_RIGID/LConn1
  Transform58/RConn1 -- x0402_H060_step_45_RIGID/LConn1
  Transform59/RConn1 -- x0402_H060_step_32_RIGID/LConn1
  Transform6/RConn1 -- x0402_H040_step_5_RIGID/LConn1
  Transform60/RConn1 -- x0402_H060_step_28_RIGID/LConn1
  Transform61/RConn1 -- x0402_H060_step_43_RIGID/LConn1
  Transform62/RConn1 -- x0402_H040_step_29_RIGID/LConn1
  Transform63/RConn1 -- x0402_H060_step_51_RIGID/LConn1
  Transform64/RConn1 -- x0402_H040_step_30_RIGID/LConn1
  Transform65/RConn1 -- x0402_H040_step_33_RIGID/LConn1
  Transform66/RConn1 -- x0402_H060_step_35_RIGID/LConn1
  Transform67/RConn1 -- x0402_H060_step_33_RIGID/LConn1
  Transform68/RConn1 -- x0402_H040_step_34_RIGID/LConn1
  Transform69/RConn1 -- x0402_H040_step_26_RIGID/LConn1
  Transform7/RConn1 -- x0402_H060_step_6_RIGID/LConn1
  Transform70/RConn1 -- x0402_H060_step_30_RIGID/LConn1
  Transform71/RConn1 -- x0402_H060_step_34_RIGID/LConn1
  Transform72/RConn1 -- x0402_H060_step_36_RIGID/LConn1
  Transform73/RConn1 -- x0402_H060_step_37_RIGID/LConn1
  Transform74/RConn1 -- x0402_H040_step_32_RIGID/LConn1
  Transform75/RConn1 -- x0402_H060_step_38_RIGID/LConn1
  Transform76/RConn1 -- x0402_H040_step_28_RIGID/LConn1
  Transform77/RConn1 -- x0402_H040_step_31_RIGID/LConn1
  Transform78/RConn1 -- x0402_H060_step_31_RIGID/LConn1
  Transform79/RConn1 -- x0402_H060_step_40_RIGID/LConn1
  Transform8/RConn1 -- x0402_H060_step_4_RIGID/LConn1
  Transform80/RConn1 -- x0402_H060_step_41_RIGID/LConn1
  Transform81/RConn1 -- x0402_H060_step_44_RIGID/LConn1
  Transform82/RConn1 -- x0402_H060_step_46_RIGID/LConn1
  Transform83/RConn1 -- x0402_H060_step_47_RIGID/LConn1
  Transform84/RConn1 -- x0402_H060_step_48_RIGID/LConn1
  Transform85/RConn1 -- x0402_H060_step_49_RIGID/LConn1
  Transform86/RConn1 -- x0402_H060_step_50_RIGID/LConn1
  Transform87/RConn1 -- x0402_H060_step_52_RIGID/LConn1
  Transform88/RConn1 -- x0402_H060_step_53_RIGID/LConn1
  Transform89/RConn1 -- x0402_H060_step_77_RIGID/LConn1
  Transform9/RConn1 -- x0402_H040_step_4_RIGID/LConn1
  Transform90/RConn1 -- x0402_H060_step_55_RIGID/LConn1
  Transform91/RConn1 -- x0402_H060_step_62_RIGID/LConn1
  Transform92/RConn1 -- x0402_H060_step_69_RIGID/LConn1
  Transform93/RConn1 -- x0402_H060_step_70_RIGID/LConn1
  Transform94/RConn1 -- x0402_H060_step_56_RIGID/LConn1
  Transform95/RConn1 -- x0402_H060_step_63_RIGID/LConn1
  Transform96/RConn1 -- x0402_H060_step_64_RIGID/LConn1
  Transform97/RConn1 -- x0402_H060_step_72_RIGID/LConn1
  Transform98/RConn1 -- x0402_H060_step_73_RIGID/LConn1
  Transform99/RConn1 -- x0402_H060_step_57_RIGID/LConn1
